simulink model "OcularMotorLabModel_2024_01_02_M21b"  (R2021b)
settings: Solver=FixedStepAuto  StartTime=tStart  StopTime=tFinal  FixedStep=0.001  RelTol=1e-3
undefined symbols (not defined in the file or in its folder): Asp, Asp1, Asp2, e0sp, gaussian, Gpc, GPos, Gsl, HeadToEye, IPD, psi, Psp1, RotFbk, SacThDeg, SatSp, sigbuilder_block, SomFbk, T1, T2, Tccanal, Tcn, Tcr, Tcsp, TCvs, tdm, tdsp1, tdsp2, tdsp3, tdv, Tsl, Tz, w
libraries: matrix_library x16, vrlib x9, simulink_extras x8, simulink x1
(part 2 of 2)

== system OcularMotorLabModel_2024_01_02_M21b/Right eye plant ==
  In1 : Inport
  Demux : Demux  Outputs=3
  Mux : Mux  Inputs=3
  Plant1 : TransferFcn  Numerator=[Tz 1]  Denominator=[T1*T2 (T1+T2) 1]
  Plant2 : TransferFcn  Numerator=[w^2]  Denominator=[1 + 2*psi*w w^2]
  Plant3 : TransferFcn  Numerator=[Tz 1]  Denominator=[T1*T2 (T1+T2) 1]
  Plant4 : TransferFcn  Numerator=[w^2]  Denominator=[1 + 2*psi*w w^2]
  Plant5 : TransferFcn  Numerator=[Tz 1]  Denominator=[T1*T2 (T1+T2) 1]
  Plant6 : TransferFcn  Numerator=[w^2]  Denominator=[1 + 2*psi*w w^2]
  Saturation : Saturate  UpperLimit=50*pi/180  LowerLimit=-50*pi/180
  Eye position : Outport
  wires:
  In1/1 -> Demux/1
  Mux/1 -> Saturation/1  "Eye position"
  Plant4/1 -> Mux/1
  Plant2/1 -> Mux/2
  Plant6/1 -> Mux/3
  Demux/1 -> Plant3/1
  Demux/2 -> Plant1/1
  Demux/3 -> Plant5/1
  Saturation/1 -> Eye position/1
  Plant3/1 -> Plant4/1
  Plant1/1 -> Plant2/1
  Plant5/1 -> Plant6/1

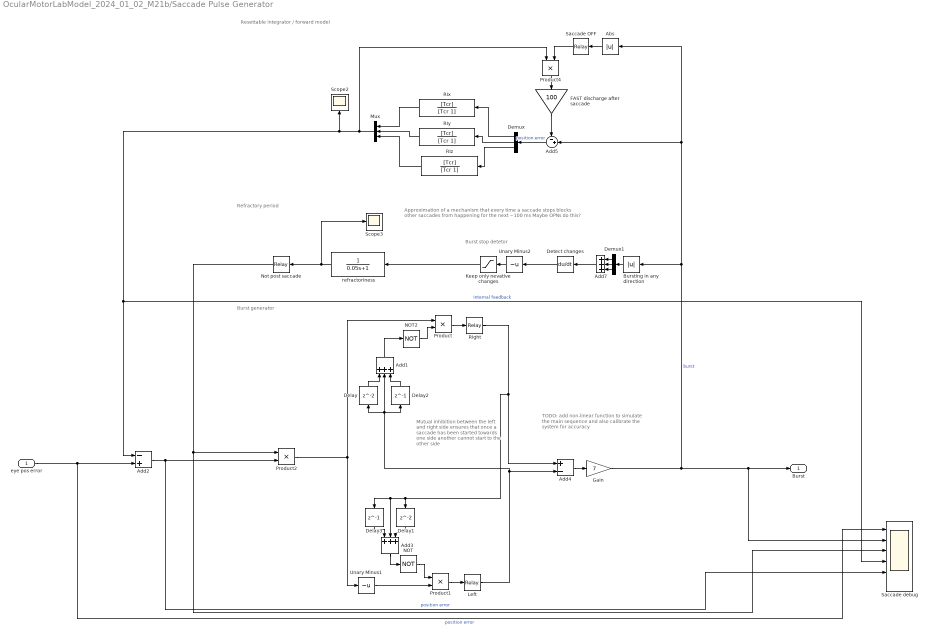
== system OcularMotorLabModel_2024_01_02_M21b/Saccade Pulse Generator ==
  note: Burst generator
  note: Resettable integrator / forward model
  note: Refractory period
  note: Burst stop detetor
  note: Mutual inhibition between the left and right side ensures that once a saccade has been started towards one side another cannot start to the other side
  note: TODO: add non-linear function to simulate the main sequence and also calibrate the system for accuracy
  note: Approximation of a mechanism that every time a saccade stops blocks other saccades from happening for the next ~100 ms
      | Maybe OPNs do this?
  eye pos error : Inport
  Abs : Abs
  Add1 : Sum  Inputs=+++
  Add2 : Sum  Inputs=-+
  Add3 : Sum  Inputs=+++
  Add4 : Sum  Inputs=+-
  Add5 : Sum  Inputs=-+|
  Add7 : Sum  Inputs=+++
  Bursting in any direction : Abs
  Delay : Delay  InitialCondition=0
  Delay1 : Delay  InitialCondition=0
  Delay2 : Delay  DelayLength=1  InitialCondition=0
  Delay3 : Delay  DelayLength=1  InitialCondition=0
  Demux : Demux  Outputs=3
  Demux1 : Demux  Outputs=3
  Detect changes : Derivative
  FAST discharge after saccade : Gain  Gain=100
  Gain : Gain  Gain=7
  Keep only nevative changes : Saturate  UpperLimit=50000000  LowerLimit=0
  Left : Relay  OnSwitchValue=SacThDeg/180*pi  OffSwitchValue=0
  Mux : Mux  Inputs=3
  NOT : Logic  Operator=NOT  IconShape=distinctive  AllPortsSameDT=off  OutDataTypeStr=boolean
  NOT2 : Logic  Operator=NOT  IconShape=distinctive  AllPortsSameDT=off  OutDataTypeStr=boolean
  Not post saccade : Relay  OnSwitchValue=1  OffSwitchValue=1  OnOutputValue=0  OffOutputValue=1
  Product{,1..2,4} (4 alike) : Product
  RIx : TransferFcn  Numerator=[Tcr]  Denominator=[Tcr 1]
  RIy : TransferFcn  Numerator=[Tcr]  Denominator=[Tcr 1]
  RIz : TransferFcn  Numerator=[Tcr]  Denominator=[Tcr 1]
  Right : Relay  OnSwitchValue=SacThDeg/180*pi  OffSwitchValue=0
  Saccade OFF : Relay  OnOutputValue=0  OffOutputValue=1
  Saccade debug : Scope  NumInputPorts=6
  Scope2 : Scope
  Scope3 : Scope
  Unary Minus1 : UnaryMinus
  Unary Minus2 : UnaryMinus
  refractoriness : TransferFcn  Numerator=1  Denominator=[0.05 1]
  Burst : Outport  VectorParamsAs1DForOutWhenUnconnected=off
  wires:
  eye pos error/1 -> Saccade debug/1, Add2/2  "position error"
  Add2/1 -> Saccade debug/5, Product2/2  "position error"
  Add7/1 -> Detect changes/1
  Detect changes/1 -> Unary Minus2/1
  Demux1/1 -> Add7/1
  Demux1/3 -> Add7/3
  Unary Minus2/1 -> Keep only nevative changes/1
  Demux1/2 -> Add7/2
  Bursting in any direction/1 -> Demux1/1
  refractoriness/1 -> Not post saccade/1, Scope3/1
  Keep only nevative changes/1 -> refractoriness/1
  Abs/1 -> Saccade OFF/1
  Product4/1 -> FAST discharge after saccade/1
  Mux/1 -> Saccade debug/4, Add2/1, Scope2/1, Product4/1  "Internal feedback"
  FAST discharge after saccade/1 -> Add5/1
  Saccade OFF/1 -> Product4/2
  Not post saccade/1 -> Saccade debug/3, Product2/1
  Add3/1 -> NOT/1
  Delay/1 -> Add1/1
  Delay2/1 -> Add1/3
  Unary Minus1/1 -> Product1/2
  Add4/1 -> Gain/1
  Product2/1 -> Product/1, Unary Minus1/1
  Add1/1 -> NOT2/1
  Product1/1 -> Left/1
  Product/1 -> Right/1
  NOT2/1 -> Product/2
  Delay1/1 -> Add3/3
  NOT/1 -> Product1/1
  Left/1 -> Add4/2, Delay2/1, Add1/2, Delay/1
  Gain/1 -> Saccade debug/2, Burst/1, Abs/1, Add5/2, Bursting in any direction/1  "burst"
  Delay3/1 -> Add3/1
  Right/1 -> Delay3/1, Add3/2, Delay1/1, Add4/1
  Demux/1 -> RIx/1
  RIy/1 -> Mux/2
  RIx/1 -> Mux/1
  Demux/3 -> RIz/1
  Demux/2 -> RIy/1
  RIz/1 -> Mux/3
  Add5/1 -> Demux/1  "position error"

== system OcularMotorLabModel_2024_01_02_M21b/Saccade velocity corollary ==
  note: Gaze holding integrator
  note: It's important for this internal model to not have a leaky integrator. Otherwise a positive feedback loop is created with retinal motion that it is not discounted but amplified post saccades.
      |
      | Haven't fully grasped it and there are still questions about the plant and the slide. But for now this seems to work ok.
  Burst : Inport
  Corollary debug : Scope  NumInputPorts=6
  Demux2 : Demux  Outputs=3
  Direct : Gain  Gain=Gpc
  Eye plant : Subsystem
  Integrator : Integrator
  "MN " : Sum  Inputs=+++  InputSameDT=on  SaturateOnIntegerOverflow=on  OutDataTypeStr=Inherit: Same as first input
  Mux2 : Mux  Inputs=3
  Pos2Vel1 : Derivative
  Position bias6 : TransferFcn  Numerator=[Gsl]  Denominator=[Tsl 1]
  Position bias7 : TransferFcn  Numerator=[Gsl]  Denominator=[Tsl 1]
  Position bias8 : TransferFcn  Numerator=[Gsl]  Denominator=[Tsl 1]
  Transport Delay : TransportDelay  DelayTime=tdv+tdm
  Out1 : Outport
  wires:
  Burst/1 -> Integrator/1, Direct/1, Demux2/1, Corollary debug/1  "Corollary input"
  Eye plant/1(Eye position) -> Pos2Vel1/1, Corollary debug/3  "Corollary eye position"
  "MN "/1 -> Eye plant/1(In1), Corollary debug/4  "Corollary integrator"
  Transport Delay/1 -> Out1/1
  Pos2Vel1/1 -> Corollary debug/2, Transport Delay/1  "Corollary eye velocity"
  Mux2/1 -> "MN "/3
  Integrator/1 -> "MN "/1
  Demux2/2 -> Position bias7/1
  Position bias8/1 -> Mux2/3
  Demux2/3 -> Position bias8/1
  Position bias6/1 -> Mux2/1
  Demux2/1 -> Position bias6/1
  Position bias7/1 -> Mux2/2
  Direct/1 -> "MN "/2

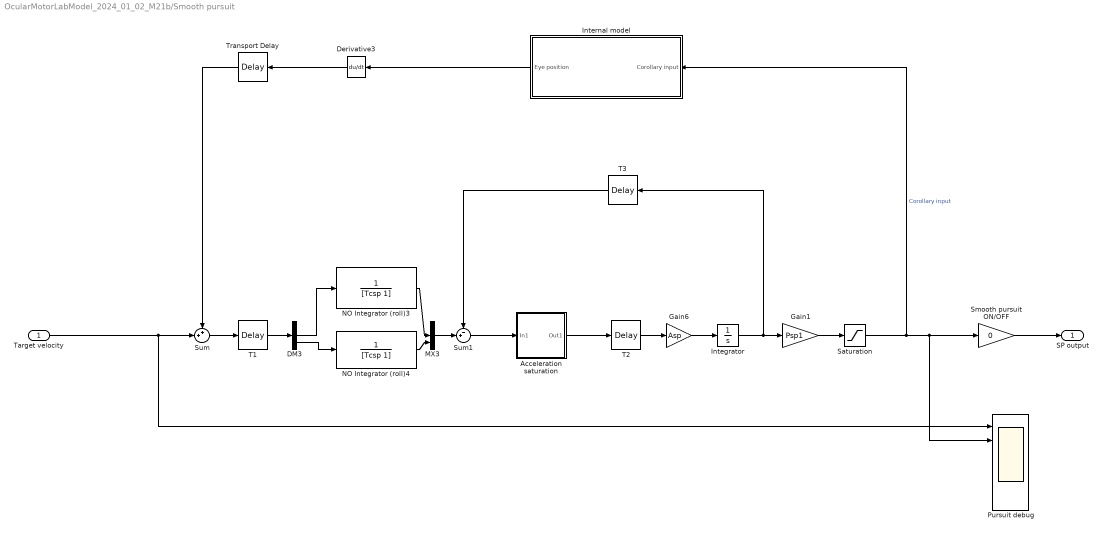
== system OcularMotorLabModel_2024_01_02_M21b/Smooth pursuit ==
  Target velocity : Inport
  Acceleration saturation : Subsystem
  DM3 : Demux  Outputs=3
  Derivative3 : Derivative
  Gain1 : Gain  Gain=Psp1
  Gain6 : Gain  Gain=Asp
  Integrator : Integrator
  Internal model : Subsystem
  MX3 : Mux  Inputs=3
  NO Integrator (roll)3 : TransferFcn  Denominator=[Tcsp 1]
  NO Integrator (roll)4 : TransferFcn  Denominator=[Tcsp 1]
  Pursuit debug : Scope  NumInputPorts=6
  Saturation : Saturate  UpperLimit=deg2rad(SatSp)  LowerLimit=-deg2rad(SatSp)
  Smooth pursuit ON/OFF : Gain  Gain=0
  Sum : Sum  Inputs=++|
  Sum1 : Sum  Inputs=-+|
  T1 : TransportDelay  DelayTime=tdsp1
  T2 : TransportDelay  DelayTime=tdsp2
  T3 : TransportDelay  DelayTime=tdsp3
  Transport Delay : TransportDelay  DelayTime=tdv+tdm
  SP output : Outport
  wires:
  Target velocity/1 -> Pursuit debug/1, Sum/2
  Sum/1 -> T1/1
  Transport Delay/1 -> Sum/1
  MX3/1 -> Sum1/2
  DM3/2 -> NO Integrator (roll)3/1
  NO Integrator (roll)3/1 -> MX3/2
  DM3/3 -> NO Integrator (roll)4/1
  NO Integrator (roll)4/1 -> MX3/3
  T1/1 -> DM3/1
  Gain6/1 -> Integrator/1
  Integrator/1 -> T3/1, Gain1/1
  T2/1 -> Gain6/1
  T3/1 -> Sum1/1
  Gain1/1 -> Saturation/1
  Smooth pursuit ON/OFF/1 -> SP output/1
  Saturation/1 -> Internal model/1(Corollary input), Pursuit debug/2, Smooth pursuit ON/OFF/1  "Corollary input"
  Derivative3/1 -> Transport Delay/1
  Internal model/1(Eye position) -> Derivative3/1
  Sum1/1 -> Acceleration saturation/1(In1)
  Acceleration saturation/1(Out1) -> T2/1

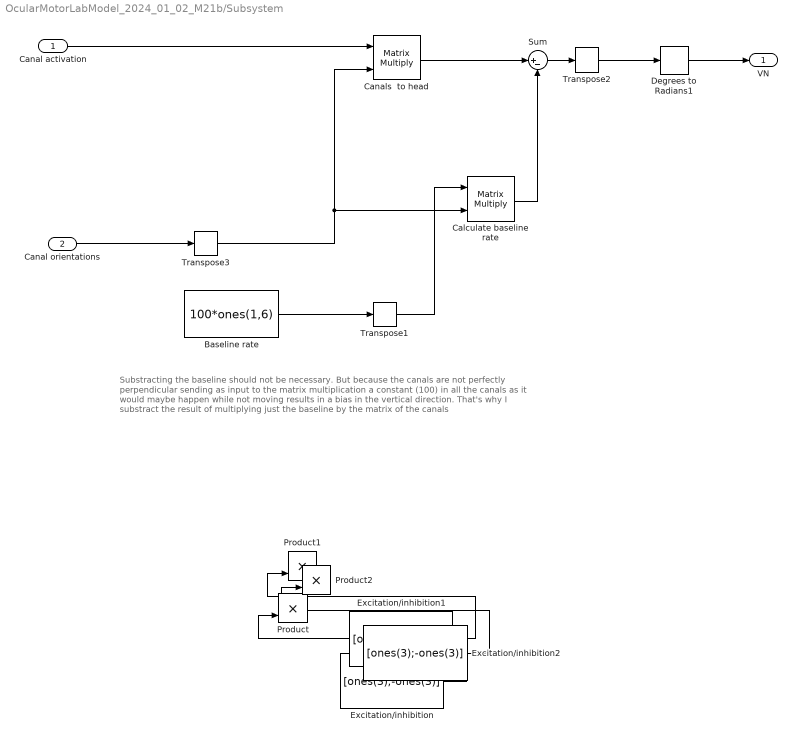
== system OcularMotorLabModel_2024_01_02_M21b/Subsystem ==
  note: Substracting the baseline should not be necessary. But because the canals are not perfectly perpendicular sending as input to the matrix multiplication a constant (100) in all the canals as it would maybe happen while not moving results in a bias in the vertical direction. That's why I substract the result of multiplying just the baseline by the matrix of the canals
  Canal activation : Inport
  Canal orientations : Inport  Port=2
  Baseline rate : Constant  Value=100*ones(1,6)
  Calculate baseline rate : Product  Multiplication=Matrix(*)
  Canals  to head : Product  Multiplication=Matrix(*)
  Degrees to Radians1 : simulink_extras/Transformations/Degrees to Radians
  Excitation/inhibition : Constant  Value=[ones(3);-ones(3)]  VectorParams1D=off
  Excitation/inhibition1 : Constant  Value=[ones(3);-ones(3)]  VectorParams1D=off
  Excitation/inhibition2 : Constant  Value=[ones(3);-ones(3)]  VectorParams1D=off
  Product : Product
  Product1 : Product
  Product2 : Product
  Sum : Sum  Inputs=|+-
  Transpose1 : matrix_library/Transpose
  Transpose2 : matrix_library/Transpose
  Transpose3 : matrix_library/Transpose
  VN : Outport
  wires:
  Sum/1 -> Transpose2/1
  Transpose2/1 -> Degrees to Radians1/1
  Transpose3/1 -> Calculate baseline rate/2, Canals  to head/2
  Excitation/inhibition/1 -> Product/2
  Excitation/inhibition1/1 -> Product1/2
  Excitation/inhibition2/1 -> Product2/2
  Canal orientations/1 -> Transpose3/1
  Canal activation/1 -> Canals  to head/1
  Baseline rate/1 -> Transpose1/1
  Calculate baseline rate/1 -> Sum/2
  Canals  to head/1 -> Sum/1
  Transpose1/1 -> Calculate baseline rate/1
  Degrees to Radians1/1 -> VN/1

== system OcularMotorLabModel_2024_01_02_M21b/Target position ==
  Bus Creator : BusCreator  Tag=Bus Creator  Inputs=3
  FromWs : FromWorkspace  Tag=STV FromWs  VariableName=tuvar
      SigBuilderData=|
      | common.afterFinalStr = 'Extrapolate'
      | common.sampleTime = 0
      | dataSet(1).timeRange = [0 88]
      | dataSet(1).name = 'Fixed streight ahead'
      | dataSet(2).timeRange = [0 88]
      | dataSet(2).name = 'Saccade Left and back'
      | dataSet(3).timeRange = [0 88]
      | dataSet(3).name = 'Saccade Right and back small'
      | dataSet(4).timeRange = [0 88]
      | dataSet(4).name = 'Saccade Up down and back'
      | dataSet(5).timeRange = [0 88]
      | dataSet(5).name = 'Horizontal smooth pursuit'
      | dataSet(6).timeRange = [0 88]
      | dataSet(6).name = 'Vergence'
      | dataSet(7).timeRange = [0 88]
      | dataSet(7).name = 'Saccade Oblique'
      | sbobj.Groups(1).Name = 'Fixed streight ahead'
      | sbobj.Groups(1).Signals(1).Name = 'tX (m - postiive forward)'
      | sbobj.Groups(1).Signals(1).XData = [0 88]
      | sbobj.Groups(1).Signals(1).YData = [1 1]
      | sbobj.Groups(1).Signals(2).Name = 'tY (m - postive to left)'
      | sbobj.Groups(1).Signals(2).XData = [0 5 35 88]
      | sbobj.Groups(1).Signals(2).YData = [0 0 0 0]
      | sbobj.Groups(1).Signals(3).Name = 'tZ (m - positive up)'
      | sbobj.Groups(1).Signals(3).XData = [0 88]
      | sbobj.Groups(1).Signals(3).YData = [0 0]
      | sbobj.Groups(1).TimeRange = [0 88]
      | sbobj.Groups(2).Name = 'Saccade Left and back'
      | sbobj.Groups(2).Signals(1).Name = 'tX (m - postiive forward)'
      | sbobj.Groups(2).Signals(1).XData = [0 88]
      | sbobj.Groups(2).Signals(1).YData = [1 1]
      | sbobj.Groups(2).Signals(2).Name = 'tY (m - postive to left)'
      | sbobj.Groups(2).Signals(2).XData = [0 5 5 25.1 25.1 88]
      | sbobj.Groups(2).Signals(2).YData = [0 0 0.5 0.5 0 0]
      | sbobj.Groups(2).Signals(3).Name = 'tZ (m - positive up)'
      | sbobj.Groups(2).Signals(3).XData = [0 88]
      | sbobj.Groups(2).Signals(3).YData = [0 0]
      | sbobj.Groups(2).TimeRange = [0 88]
      | sbobj.Groups(3).Name = 'Saccade Right and back small'
      | sbobj.Groups(3).Signals(1).Name = 'tX (m - postiive forward)'
      | sbobj.Groups(3).Signals(1).XData = [0 88]
      | sbobj.Groups(3).Signals(1).YData = [1 1]
      | sbobj.Groups(3).Signals(2).Name = 'tY (m - postive to left)'
      | sbobj.Groups(3).Signals(2).XData = [0 5 5 35 35 88]
      | sbobj.Groups(3).Signals(2).YData = [0 0 0.02 0.02 0 0]
      | sbobj.Groups(3).Signals(3).Name = 'tZ (m - positive up)'
      | sbobj.Groups(3).Signals(3).XData = [0 88]
      | sbobj.Groups(3).Signals(3).YData = [0 0]
      | sbobj.Groups(3).TimeRange = [0 88]
      | sbobj.Groups(4).Name = 'Saccade Up down and back'
      | sbobj.Groups(4).Signals(1).Name = 'tX (m - postiive forward)'
      | sbobj.Groups(4).Signals(1).XData = [0 88]
      | sbobj.Groups(4).Signals(1).YData = [1 1]
      | sbobj.Groups(4).Signals(2).Name = 'tY (m - postive to left)'
      | sbobj.Groups(4).Signals(2).XData = [0 5 35 88]
      | sbobj.Groups(4).Signals(2).YData = [0 0 0 0]
      | sbobj.Groups(4).Signals(3).Name = 'tZ (m - positive up)'
      | sbobj.Groups(4).Signals(3).XData = [0 10 10 13.1 13.1 88]
      | sbobj.Groups(4).Signals(3).YData = [0 0 0.5 0.5 0 0]
      | sbobj.Groups(4).TimeRange = [0 88]
      | sbobj.Groups(5).Name = 'Horizontal smooth pursuit'
      | sbobj.Groups(5).Signals(1).Name = 'tX (m - postiive forward)'
      | sbobj.Groups(5).Signals(1).XData = [0 88]
      | sbobj.Groups(5).Signals(1).YData = [1 1]
      | sbobj.Groups(5).Signals(2).Name = 'tY (m - postive to left)'
      | sbobj.Groups(5).Signals(2).XData = [0 10 20 20 88]
      | sbobj.Groups(5).Signals(2).YData = [0 0 0.5 0 0]
      | sbobj.Groups(5).Signals(3).Name = 'tZ (m - positive up)'
      | sbobj.Groups(5).Signals(3).XData = [0 10 20 88]
      | sbobj.Groups(5).Signals(3).YData = [0 0 0 0]
      | sbobj.Groups(5).TimeRange = [0 88]
      | sbobj.Groups(6).Name = 'Vergence'
      | sbobj.Groups(6).Signals(1).Name = 'tX (m - postiive forward)'
      | sbobj.Groups(6).Signals(1).XData = [0 10 10 20 20 30 30 40 40 50 50 60 60 70 70 80 80 88]
      | sbobj.Groups(6).Signals(1).YData = [1.25 1.25 0.25 0.25 1.25 1.25 0.25 0.25 1.25 1.25 0.25 0.25 1.25 1.25 0.25 0.25 1.25 1.25]
      | sbobj.Groups(6).Signals(2).Name = 'tY (m - postive to left)'
      | sbobj.Groups(6).Signals(2).XData = [0 5 25.1 88]
      | sbobj.Groups(6).Signals(2).YData = [0 0 0 0]
      | sbobj.Groups(6).Signals(3).Name = 'tZ (m - positive up)'
      | sbobj.Groups(6).Signals(3).XData = [0 88]
      | sbobj.Groups(6).Signals(3).YData = [0 0]
      | sbobj.Groups(6).TimeRange = [0 88]
      | sbobj.Groups(7).Name = 'Saccade Oblique'
      | sbobj.Groups(7).Signals(1).Name = 'tX (m - postiive forward)'
      | sbobj.Groups(7).Signals(1).XData = [0 88]
      | sbobj.Groups(7).Signals(1).YData = [1 1]
      | sbobj.Groups(7).Signals(2).Name = 'tY (m - postive to left)'
      | sbobj.Groups(7).Signals(2).XData = [0 10 10 20 20 88]
      | sbobj.Groups(7).Signals(2).YData = [0 0 0.5 0.5 0 0]
      | sbobj.Groups(7).Signals(3).Name = 'tZ (m - positive up)'
      | sbobj.Groups(7).Signals(3).XData = [0 10 10 20 20 88]
      | sbobj.Groups(7).Signals(3).YData = [0 0 0.5 0.5 0 0]
      | sbobj.Groups(7).TimeRange = [0 88]
  Subsystem : Subsystem
  Bus : Outport
  wires:
  FromWs/1 -> Subsystem/1(In1)
  Subsystem/1(tX (m - postiive forward)) -> Bus Creator/1  "tX (m - postiive forward)"
  Subsystem/2(tY (m - postive to left)) -> Bus Creator/2  "tY (m - postive to left)"
  Subsystem/3(tZ (m - positive up)) -> Bus Creator/3  "tZ (m - positive up)"
  Bus Creator/1 -> Bus/1

== system OcularMotorLabModel_2024_01_02_M21b/Velocity storage ==
  In1 : Inport
  DM : Demux  Outputs=3
  IA Integrator (pitch) : TransferFcn  Numerator=1  Denominator=[TCvs 1]
  MX : Mux  Inputs=3
  NO Integrator (roll) : TransferFcn  Numerator=1  Denominator=[TCvs 1]
  RC Integrator (yaw) : TransferFcn  Numerator=1  Denominator=[TCvs 1]
  Out1 : Outport
  wires:
  MX/1 -> Out1/1
  DM/3 -> RC Integrator (yaw)/1
  RC Integrator (yaw)/1 -> MX/3
  IA Integrator (pitch)/1 -> MX/2
  NO Integrator (roll)/1 -> MX/1
  DM/1 -> NO Integrator (roll)/1
  In1/1 -> DM/1
  DM/2 -> IA Integrator (pitch)/1

== system OcularMotorLabModel_2024_01_02_M21b/Vergence ==
  Target distance estimate (Diopters) : Inport
  Vergence error : Inport  Port=2
  Transfer Fcn : TransferFcn  Denominator=[0.1 1]
  Vergence on/off : Gain
  Vergence : Outport
  Accomodation : Outport  Port=2
  wires:
  Vergence on/off/1 -> Vergence/1
  Vergence error/1 -> Transfer Fcn/1
  Target distance estimate (Diopters)/1 -> ?
  Transfer Fcn/1 -> Vergence on/off/1

== system OcularMotorLabModel_2024_01_02_M21b/Vergence (distance) corollary ==
  Motor output : Inport
  Asin5 : Trigonometry  Operator=tan
  Corollary debug : Scope  NumInputPorts=6
  Divide3 : Product  Inputs=*/
  Eye plant : Subsystem
  IPD : Constant  Value=IPD/2
  Diopters : Outport
  wires:
  Motor output/1 -> Corollary debug/1, Eye plant/1(Motor output)  "Corollary input"
  Eye plant/1(Eye position) -> Corollary debug/2, Asin5/1  "Corollary eye position"
  Divide3/1 -> Diopters/1, Corollary debug/3
  IPD/1 -> Divide3/2
  Asin5/1 -> Divide3/1

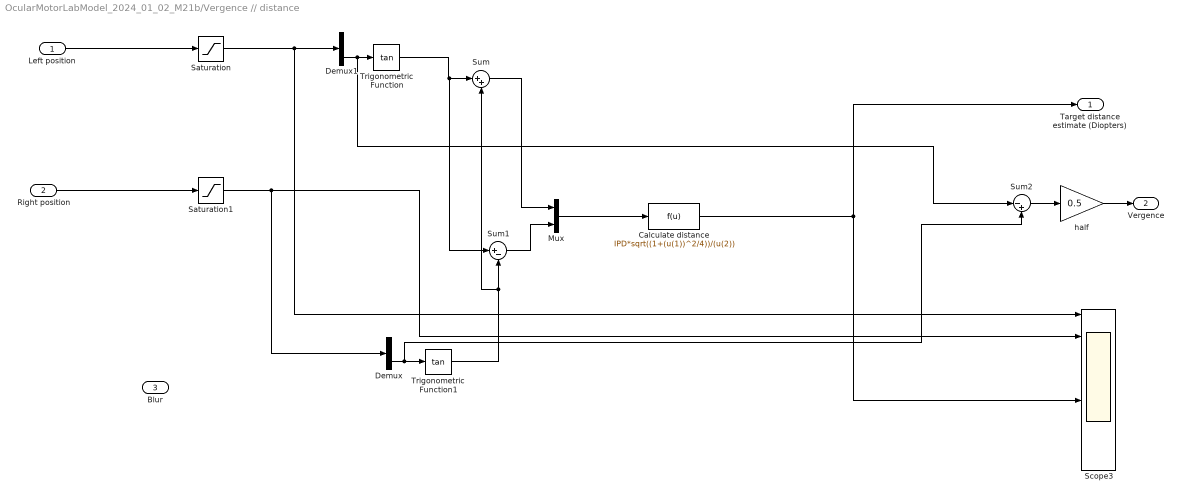
== system OcularMotorLabModel_2024_01_02_M21b/Vergence // distance ==
  Left position : Inport
  Right position : Inport  Port=2
  Blur : Inport  Port=3
  Calculate distance : Fcn  Expr=IPD*sqrt((1+(u(1))^2/4))/(u(2))
  Demux : Demux  Outputs=3
  Demux1 : Demux  Outputs=3
  Mux : Mux  Inputs=2
  Saturation : Saturate  UpperLimit=50*pi/180  LowerLimit=-50*pi/180
  Saturation1 : Saturate  UpperLimit=50*pi/180  LowerLimit=-50*pi/180
  Scope3 : Scope  NumInputPorts=8
  Sum : Sum  Inputs=|++
  Sum1 : Sum  Inputs=|+-
  Sum2 : Sum  Inputs=|-+
  Trigonometric Function : Trigonometry  Operator=tan
  Trigonometric Function1 : Trigonometry  Operator=tan
  half : Gain  Gain=0.5
  Target distance estimate (Diopters) : Outport
  Vergence : Outport  Port=2
  wires:
  Left position/1 -> Saturation/1
  Right position/1 -> Saturation1/1
  Mux/1 -> Calculate distance/1
  Demux1/3 -> Sum2/1, Trigonometric Function/1
  Demux/3 -> Sum2/2, Trigonometric Function1/1
  Calculate distance/1 -> Scope3/5, Target distance estimate (Diopters)/1
  Trigonometric Function/1 -> Sum1/1, Sum/1
  Trigonometric Function1/1 -> Sum/2, Sum1/2
  Sum/1 -> Mux/1
  Sum1/1 -> Mux/2
  Sum2/1 -> half/1
  Saturation/1 -> Scope3/1, Demux1/1
  Saturation1/1 -> Scope3/2, Demux/1
  half/1 -> Vergence/1

== system OcularMotorLabModel_2024_01_02_M21b/Version ==
  Left : Inport
  Right : Inport  Port=2
  Gain : Gain  Gain=1/2
  Saccade debug : Scope  NumInputPorts=6
  Sum : Sum  Inputs=+|+
  Out1 : Outport
  wires:
  Gain/1 -> Saccade debug/3, Out1/1
  Sum/1 -> Gain/1
  Left/1 -> Saccade debug/1, Sum/1
  Right/1 -> Saccade debug/2, Sum/2

== system OcularMotorLabModel_2024_01_02_M21b/Version Position corollary ==
  Motor output : Inport
  Asin1 : Trigonometry
  Asin2 : Trigonometry  Operator=cos
  Asin3 : Trigonometry  Operator=cos
  Asin4 : Trigonometry
  Corollary debug : Scope  NumInputPorts=6
  Demux3 : Demux  Outputs=3
  Divide1 : Product  Inputs=**
  Divide2 : Product  Inputs=**
  Eye plant : Subsystem
  Mux3 : Mux  Inputs=3
  Out1 : Outport
  wires:
  Eye plant/1(Eye position) -> Demux3/1, Corollary debug/3  "Corollary eye position"
  Divide1/1 -> Mux3/1
  Asin1/1 -> Mux3/3
  Demux3/2 -> Asin3/1, Asin1/1
  Divide2/1 -> Mux3/2
  Asin3/1 -> Divide2/2, Divide1/2
  Asin2/1 -> Divide1/1
  Asin4/1 -> Divide2/1
  Demux3/3 -> Asin2/1, Asin4/1
  Mux3/1 -> Corollary debug/5, Out1/1  "Step"
  Motor output/1 -> Eye plant/1(Motor output)  "Corollary input"

== system OcularMotorLabModel_2024_01_02_M21b/Visual World Extrinsic Orientation ==
  Bus Creator : BusCreator  Tag=Bus Creator  Inputs=3
  FromWs : FromWorkspace  Tag=STV FromWs  VariableName=tuvar
      SigBuilderData=|
      | common.afterFinalStr = 'Extrapolate'
      | common.sampleTime = 0
      | dataSet(1).timeRange = [0 60]
      | dataSet(1).name = 'Zeros'
      | dataSet(2).timeRange = [0 60]
      | dataSet(2).name = 'Roll 0.2 Hz'
      | dataSet(3).timeRange = [0 60]
      | dataSet(3).name = 'Roll 0.1 Hz'
      | dataSet(4).timeRange = [0 60]
      | dataSet(4).name = 'Roll 0.05 Hz'
      | dataSet(5).timeRange = [0 60]
      | dataSet(5).name = 'Roll 0.2 Hz IA'
      | dataSet(6).timeRange = [0 60]
      | dataSet(6).name = 'Roll 0.1 Hz IA'
      | dataSet(7).timeRange = [0 60]
      | dataSet(7).name = 'Roll 0.05 Hz IA'
      | dataSet(8).timeRange = [0 60]
      | dataSet(8).name = 'Roll 0.2 Hz RC'
      | dataSet(9).timeRange = [0 60]
      | dataSet(9).name = 'Roll 0.1 Hz RC'
      | dataSet(10).timeRange = [0 60]
      | dataSet(10).name = 'Roll 0.05 Hz RC'
      | dataSet(11).timeRange = [0 60]
      | dataSet(11).name = 'SimpleSims'
      | sbobj.Groups(1).Name = 'Zeros'
      | sbobj.Groups(1).Signals(1).Name = 'N-O (roll)'
      | sbobj.Groups(1).Signals(1).XData = [0 60]
      | sbobj.Groups(1).Signals(1).YData = [0 0]
      | sbobj.Groups(1).Signals(2).Name = 'I-A (pitch)'
      | sbobj.Groups(1).Signals(2).XData = [0 60]
      | sbobj.Groups(1).Signals(2).YData = [0 0]
      | sbobj.Groups(1).Signals(3).Name = 'R-C (yaw)'
      | sbobj.Groups(1).Signals(3).XData = [0 60]
      | sbobj.Groups(1).Signals(3).YData = [0 0]
      | sbobj.Groups(1).TimeRange = [0 60]
      | sbobj.Groups(2).Name = 'Roll 0.2 Hz'
      | sbobj.Groups(2).Signals(1).Name = 'N-O (roll)'
      | sbobj.Groups(2).Signals(1).XData = [0 0.00500500500501 0.01001001001 0.015015015015 0.02002002002 0.025025025025 0.03003003003 0.035035035035 0.04004004004 0.045045045045 0.0500500500501 0.0550550550551 ... (11989 elements, 1x11989)]
      | sbobj.Groups(2).Signals(1).YData = [0 0.125788666321 0.251572356775 0.377346095689 0.503104907788 0.628843818382 0.754557853574 0.880242040448 1.00589140727 1.13150098368 1.25706580089 1.3825808919 ... (11989 elements, 1x11989)]
      | sbobj.Groups(2).Signals(2).Name = 'I-A (pitch)'
      | sbobj.Groups(2).Signals(2).XData = [0 60]
      | sbobj.Groups(2).Signals(2).YData = [0 0]
      | sbobj.Groups(2).Signals(3).Name = 'R-C (yaw)'
      | sbobj.Groups(2).Signals(3).XData = [0 60]
      | sbobj.Groups(2).Signals(3).YData = [0 0]
      | sbobj.Groups(2).TimeRange = [0 60]
      | sbobj.Groups(3).Name = 'Roll 0.1 Hz'
      | sbobj.Groups(3).Signals(1).Name = 'N-O (roll)'
      | sbobj.Groups(3).Signals(1).XData = [0 0.01001001001 0.02002002002 0.03003003003 0.04004004004 0.0500500500501 0.0600600600601 0.0700700700701 0.0800800800801 0.0900900900901 0.1001001001 0.11011011011 ... (5995 elements, 1x5995)]
      | sbobj.Groups(3).Signals(1).YData = [0 0.125788666321 0.251572356775 0.377346095689 0.503104907788 0.628843818382 0.754557853574 0.880242040448 1.00589140727 1.13150098368 1.25706580089 1.3825808919 ... (5995 elements, 1x5995)]
      | sbobj.Groups(3).Signals(2).Name = 'I-A (pitch)'
      | sbobj.Groups(3).Signals(2).XData = [0 60]
      | sbobj.Groups(3).Signals(2).YData = [0 0]
      | sbobj.Groups(3).Signals(3).Name = 'R-C (yaw)'
      | sbobj.Groups(3).Signals(3).XData = [0 60]
      | sbobj.Groups(3).Signals(3).YData = [0 0]
      | sbobj.Groups(3).TimeRange = [0 60]
      | sbobj.Groups(4).Name = 'Roll 0.05 Hz'
      | sbobj.Groups(4).Signals(1).Name = 'N-O (roll)'
      | sbobj.Groups(4).Signals(1).XData = [0 0.02002002002 0.04004004004 0.0600600600601 0.0800800800801 0.1001001001 0.12012012012 0.14014014014 0.16016016016 0.18018018018 0.2002002002 0.22022022022 ... (2998 elements, 1x2998)]
      | sbobj.Groups(4).Signals(1).YData = [0 0.125788666321 0.251572356775 0.377346095689 0.503104907788 0.628843818382 0.754557853574 0.880242040448 1.00589140727 1.13150098368 1.25706580089 1.3825808919 ... (2998 elements, 1x2998)]
      | sbobj.Groups(4).Signals(2).Name = 'I-A (pitch)'
      | sbobj.Groups(4).Signals(2).XData = [0 60]
      | sbobj.Groups(4).Signals(2).YData = [0 0]
      | sbobj.Groups(4).Signals(3).Name = 'R-C (yaw)'
      | sbobj.Groups(4).Signals(3).XData = [0 60]
      | sbobj.Groups(4).Signals(3).YData = [0 0]
      | sbobj.Groups(4).TimeRange = [0 60]
      | sbobj.Groups(5).Name = 'Roll 0.2 Hz IA'
      | sbobj.Groups(5).Signals(1).Name = 'N-O (roll)'
      | sbobj.Groups(5).Signals(1).XData = [0 60]
      | sbobj.Groups(5).Signals(1).YData = [0 0]
      | sbobj.Groups(5).Signals(2).Name = 'I-A (pitch)'
      | sbobj.Groups(5).Signals(2).XData = [0 0.00500500500501 0.01001001001 0.015015015015 0.02002002002 0.025025025025 0.03003003003 0.035035035035 0.04004004004 0.045045045045 0.0500500500501 0.0550550550551 ... (11989 elements, 1x11989)]
      | sbobj.Groups(5).Signals(2).YData = [0 0.125788666321 0.251572356775 0.377346095689 0.503104907788 0.628843818382 0.754557853574 0.880242040448 1.00589140727 1.13150098368 1.25706580089 1.3825808919 ... (11989 elements, 1x11989)]
      | sbobj.Groups(5).Signals(3).Name = 'R-C (yaw)'
      | sbobj.Groups(5).Signals(3).XData = [0 60]
      | sbobj.Groups(5).Signals(3).YData = [0 0]
      | sbobj.Groups(5).TimeRange = [0 60]
      | sbobj.Groups(6).Name = 'Roll 0.1 Hz IA'
      | sbobj.Groups(6).Signals(1).Name = 'N-O (roll)'
      | sbobj.Groups(6).Signals(1).XData = [0 60]
      | sbobj.Groups(6).Signals(1).YData = [0 0]
      | sbobj.Groups(6).Signals(2).Name = 'I-A (pitch)'
      | sbobj.Groups(6).Signals(2).XData = [0 0.01001001001 0.02002002002 0.03003003003 0.04004004004 0.0500500500501 0.0600600600601 0.0700700700701 0.0800800800801 0.0900900900901 0.1001001001 0.11011011011 ... (5995 elements, 1x5995)]
      | sbobj.Groups(6).Signals(2).YData = [0 0.125788666321 0.251572356775 0.377346095689 0.503104907788 0.628843818382 0.754557853574 0.880242040448 1.00589140727 1.13150098368 1.25706580089 1.3825808919 ... (5995 elements, 1x5995)]
      | sbobj.Groups(6).Signals(3).Name = 'R-C (yaw)'
      | sbobj.Groups(6).Signals(3).XData = [0 60]
      | sbobj.Groups(6).Signals(3).YData = [0 0]
      | sbobj.Groups(6).TimeRange = [0 60]
      | sbobj.Groups(7).Name = 'Roll 0.05 Hz IA'
      | sbobj.Groups(7).Signals(1).Name = 'N-O (roll)'
      | sbobj.Groups(7).Signals(1).XData = [0 60]
      | sbobj.Groups(7).Signals(1).YData = [0 0]
      | sbobj.Groups(7).Signals(2).Name = 'I-A (pitch)'
      | sbobj.Groups(7).Signals(2).XData = [0 0.02002002002 0.04004004004 0.0600600600601 0.0800800800801 0.1001001001 0.12012012012 0.14014014014 0.16016016016 0.18018018018 0.2002002002 0.22022022022 ... (2998 elements, 1x2998)]
      | sbobj.Groups(7).Signals(2).YData = [0 0.125788666321 0.251572356775 0.377346095689 0.503104907788 0.628843818382 0.754557853574 0.880242040448 1.00589140727 1.13150098368 1.25706580089 1.3825808919 ... (2998 elements, 1x2998)]
      | sbobj.Groups(7).Signals(3).Name = 'R-C (yaw)'
      | sbobj.Groups(7).Signals(3).XData = [0 60]
      | sbobj.Groups(7).Signals(3).YData = [0 0]
      | sbobj.Groups(7).TimeRange = [0 60]
      | sbobj.Groups(8).Name = 'Roll 0.2 Hz RC'
      | sbobj.Groups(8).Signals(1).Name = 'N-O (roll)'
      | sbobj.Groups(8).Signals(1).XData = [0 60]
      | sbobj.Groups(8).Signals(1).YData = [0 0]
      | sbobj.Groups(8).Signals(2).Name = 'I-A (pitch)'
      | sbobj.Groups(8).Signals(2).XData = [0 60]
      | sbobj.Groups(8).Signals(2).YData = [0 0]
      | sbobj.Groups(8).Signals(3).Name = 'R-C (yaw)'
      | sbobj.Groups(8).Signals(3).XData = [0 0.00500500500501 0.01001001001 0.015015015015 0.02002002002 0.025025025025 0.03003003003 0.035035035035 0.04004004004 0.045045045045 0.0500500500501 0.0550550550551 ... (11989 elements, 1x11989)]
      | sbobj.Groups(8).Signals(3).YData = [0 0.125788666321 0.251572356775 0.377346095689 0.503104907788 0.628843818382 0.754557853574 0.880242040448 1.00589140727 1.13150098368 1.25706580089 1.3825808919 ... (11989 elements, 1x11989)]
      | sbobj.Groups(8).TimeRange = [0 60]
      | sbobj.Groups(9).Name = 'Roll 0.1 Hz RC'
      | sbobj.Groups(9).Signals(1).Name = 'N-O (roll)'
      | sbobj.Groups(9).Signals(1).XData = [0 60]
      | sbobj.Groups(9).Signals(1).YData = [0 0]
      | sbobj.Groups(9).Signals(2).Name = 'I-A (pitch)'
      | sbobj.Groups(9).Signals(2).XData = [0 60]
      | sbobj.Groups(9).Signals(2).YData = [0 0]
      | sbobj.Groups(9).Signals(3).Name = 'R-C (yaw)'
      | sbobj.Groups(9).Signals(3).XData = [0 0.01001001001 0.02002002002 0.03003003003 0.04004004004 0.0500500500501 0.0600600600601 0.0700700700701 0.0800800800801 0.0900900900901 0.1001001001 0.11011011011 ... (5995 elements, 1x5995)]
      | sbobj.Groups(9).Signals(3).YData = [0 0.125788666321 0.251572356775 0.377346095689 0.503104907788 0.628843818382 0.754557853574 0.880242040448 1.00589140727 1.13150098368 1.25706580089 1.3825808919 ... (5995 elements, 1x5995)]
      | sbobj.Groups(9).TimeRange = [0 60]
      | sbobj.Groups(10).Name = 'Roll 0.05 Hz RC'
      | sbobj.Groups(10).Signals(1).Name = 'N-O (roll)'
      | sbobj.Groups(10).Signals(1).XData = [0 60]
      | sbobj.Groups(10).Signals(1).YData = [0 0]
      | sbobj.Groups(10).Signals(2).Name = 'I-A (pitch)'
      | sbobj.Groups(10).Signals(2).XData = [0 60]
      | sbobj.Groups(10).Signals(2).YData = [0 0]
      | sbobj.Groups(10).Signals(3).Name = 'R-C (yaw)'
      | sbobj.Groups(10).Signals(3).XData = [0 0.02002002002 0.04004004004 0.0600600600601 0.0800800800801 0.1001001001 0.12012012012 0.14014014014 0.16016016016 0.18018018018 0.2002002002 0.22022022022 ... (2998 elements, 1x2998)]
      | sbobj.Groups(10).Signals(3).YData = [0 0.125788666321 0.251572356775 0.377346095689 0.503104907788 0.628843818382 0.754557853574 0.880242040448 1.00589140727 1.13150098368 1.25706580089 1.3825808919 ... (2998 elements, 1x2998)]
      | sbobj.Groups(10).TimeRange = [0 60]
      | sbobj.Groups(11).Name = 'SimpleSims'
      | sbobj.Groups(11).Signals(1).Name = 'N-O (roll)'
      | sbobj.Groups(11).Signals(1).XData = [0 0.01 0.02 0.03 0.04 0.05 0.06 0.07 0.08 0.09 0.1 0.11 ... (6001 elements, 1x6001)]
      | sbobj.Groups(11).Signals(1).YData = [0 0.0628317497176 0.125662879311 0.188492768663 0.251320797667 0.314146346236 0.376968794308 0.43978752185 0.502601908867 0.565411335405 0.628215181563 0.691012827489 ... (6001 elements, 1x6001)]
      | sbobj.Groups(11).Signals(2).Name = 'I-A (pitch)'
      | sbobj.Groups(11).Signals(2).XData = [0 5 35 60]
      | sbobj.Groups(11).Signals(2).YData = [0 0 0 0]
      | sbobj.Groups(11).Signals(3).Name = 'R-C (yaw)'
      | sbobj.Groups(11).Signals(3).XData = [0 5 35 60]
      | sbobj.Groups(11).Signals(3).YData = [0 0 0 0]
      | sbobj.Groups(11).TimeRange = [0 60]
  Subsystem : Subsystem
  Bus : Outport
  wires:
  FromWs/1 -> Subsystem/1(In1)
  Subsystem/1(N-O (roll)) -> Bus Creator/1  "N-O (roll)"
  Subsystem/2(I-A (pitch)) -> Bus Creator/2  "I-A (pitch)"
  Subsystem/3(R-C (yaw)) -> Bus Creator/3  "R-C (yaw)"
  Bus Creator/1 -> Bus/1

== system OcularMotorLabModel_2024_01_02_M21b/Visual World Extrinsic velocity ==
  Bus Creator : BusCreator  Tag=Bus Creator  Inputs=3
  FromWs : FromWorkspace  Tag=STV FromWs  VariableName=tuvar
      SigBuilderData=|
      | common.afterFinalStr = 'Extrapolate'
      | common.sampleTime = 0
      | dataSet(1).timeRange = [0 60]
      | dataSet(1).name = 'Zeros'
      | dataSet(2).timeRange = [0 60]
      | dataSet(2).name = 'Roll 0.2 Hz'
      | dataSet(3).timeRange = [0 60]
      | dataSet(3).name = 'Roll 0.1 Hz'
      | dataSet(4).timeRange = [0 60]
      | dataSet(4).name = 'Roll 0.05 Hz'
      | dataSet(5).timeRange = [0 60]
      | dataSet(5).name = 'Roll 0.2 Hz IA'
      | dataSet(6).timeRange = [0 60]
      | dataSet(6).name = 'Roll 0.1 Hz IA'
      | dataSet(7).timeRange = [0 60]
      | dataSet(7).name = 'Roll 0.05 Hz IA'
      | dataSet(8).timeRange = [0 60]
      | dataSet(8).name = 'Roll 0.2 Hz RC'
      | dataSet(9).timeRange = [0 60]
      | dataSet(9).name = 'Roll 0.1 Hz RC'
      | dataSet(10).timeRange = [0 60]
      | dataSet(10).name = 'Roll 0.05 Hz RC'
      | dataSet(11).timeRange = [0 60]
      | dataSet(11).name = 'SimpleSims'
      | dataSet(12).timeRange = [0 60]
      | dataSet(12).name = 'YawOKN30degs'
      | sbobj.Groups(1).Name = 'Zeros'
      | sbobj.Groups(1).Signals(1).Name = 'N-O (roll)'
      | sbobj.Groups(1).Signals(1).XData = [0 60]
      | sbobj.Groups(1).Signals(1).YData = [0 0]
      | sbobj.Groups(1).Signals(2).Name = 'I-A (pitch)'
      | sbobj.Groups(1).Signals(2).XData = [0 60]
      | sbobj.Groups(1).Signals(2).YData = [0 0]
      | sbobj.Groups(1).Signals(3).Name = 'R-C (yaw)'
      | sbobj.Groups(1).Signals(3).XData = [0 60]
      | sbobj.Groups(1).Signals(3).YData = [0 0]
      | sbobj.Groups(1).TimeRange = [0 60]
      | sbobj.Groups(2).Name = 'Roll 0.2 Hz'
      | sbobj.Groups(2).Signals(1).Name = 'N-O (roll)'
      | sbobj.Groups(2).Signals(1).XData = [0 0.00500500500501 0.01001001001 0.015015015015 0.02002002002 0.025025025025 0.03003003003 0.035035035035 0.04004004004 0.045045045045 0.0500500500501 0.0550550550551 ... (11989 elements, 1x11989)]
      | sbobj.Groups(2).Signals(1).YData = [0 0.125788666321 0.251572356775 0.377346095689 0.503104907788 0.628843818382 0.754557853574 0.880242040448 1.00589140727 1.13150098368 1.25706580089 1.3825808919 ... (11989 elements, 1x11989)]
      | sbobj.Groups(2).Signals(2).Name = 'I-A (pitch)'
      | sbobj.Groups(2).Signals(2).XData = [0 60]
      | sbobj.Groups(2).Signals(2).YData = [0 0]
      | sbobj.Groups(2).Signals(3).Name = 'R-C (yaw)'
      | sbobj.Groups(2).Signals(3).XData = [0 60]
      | sbobj.Groups(2).Signals(3).YData = [0 0]
      | sbobj.Groups(2).TimeRange = [0 60]
      | sbobj.Groups(3).Name = 'Roll 0.1 Hz'
      | sbobj.Groups(3).Signals(1).Name = 'N-O (roll)'
      | sbobj.Groups(3).Signals(1).XData = [0 0.01001001001 0.02002002002 0.03003003003 0.04004004004 0.0500500500501 0.0600600600601 0.0700700700701 0.0800800800801 0.0900900900901 0.1001001001 0.11011011011 ... (5995 elements, 1x5995)]
      | sbobj.Groups(3).Signals(1).YData = [0 0.125788666321 0.251572356775 0.377346095689 0.503104907788 0.628843818382 0.754557853574 0.880242040448 1.00589140727 1.13150098368 1.25706580089 1.3825808919 ... (5995 elements, 1x5995)]
      | sbobj.Groups(3).Signals(2).Name = 'I-A (pitch)'
      | sbobj.Groups(3).Signals(2).XData = [0 60]
      | sbobj.Groups(3).Signals(2).YData = [0 0]
      | sbobj.Groups(3).Signals(3).Name = 'R-C (yaw)'
      | sbobj.Groups(3).Signals(3).XData = [0 60]
      | sbobj.Groups(3).Signals(3).YData = [0 0]
      | sbobj.Groups(3).TimeRange = [0 60]
      | sbobj.Groups(4).Name = 'Roll 0.05 Hz'
      | sbobj.Groups(4).Signals(1).Name = 'N-O (roll)'
      | sbobj.Groups(4).Signals(1).XData = [0 0.02002002002 0.04004004004 0.0600600600601 0.0800800800801 0.1001001001 0.12012012012 0.14014014014 0.16016016016 0.18018018018 0.2002002002 0.22022022022 ... (2998 elements, 1x2998)]
      | sbobj.Groups(4).Signals(1).YData = [0 0.125788666321 0.251572356775 0.377346095689 0.503104907788 0.628843818382 0.754557853574 0.880242040448 1.00589140727 1.13150098368 1.25706580089 1.3825808919 ... (2998 elements, 1x2998)]
      | sbobj.Groups(4).Signals(2).Name = 'I-A (pitch)'
      | sbobj.Groups(4).Signals(2).XData = [0 60]
      | sbobj.Groups(4).Signals(2).YData = [0 0]
      | sbobj.Groups(4).Signals(3).Name = 'R-C (yaw)'
      | sbobj.Groups(4).Signals(3).XData = [0 60]
      | sbobj.Groups(4).Signals(3).YData = [0 0]
      | sbobj.Groups(4).TimeRange = [0 60]
      | sbobj.Groups(5).Name = 'Roll 0.2 Hz IA'
      | sbobj.Groups(5).Signals(1).Name = 'N-O (roll)'
      | sbobj.Groups(5).Signals(1).XData = [0 60]
      | sbobj.Groups(5).Signals(1).YData = [0 0]
      | sbobj.Groups(5).Signals(2).Name = 'I-A (pitch)'
      | sbobj.Groups(5).Signals(2).XData = [0 0.00500500500501 0.01001001001 0.015015015015 0.02002002002 0.025025025025 0.03003003003 0.035035035035 0.04004004004 0.045045045045 0.0500500500501 0.0550550550551 ... (11989 elements, 1x11989)]
      | sbobj.Groups(5).Signals(2).YData = [0 0.125788666321 0.251572356775 0.377346095689 0.503104907788 0.628843818382 0.754557853574 0.880242040448 1.00589140727 1.13150098368 1.25706580089 1.3825808919 ... (11989 elements, 1x11989)]
      | sbobj.Groups(5).Signals(3).Name = 'R-C (yaw)'
      | sbobj.Groups(5).Signals(3).XData = [0 60]
      | sbobj.Groups(5).Signals(3).YData = [0 0]
      | sbobj.Groups(5).TimeRange = [0 60]
      | sbobj.Groups(6).Name = 'Roll 0.1 Hz IA'
      | sbobj.Groups(6).Signals(1).Name = 'N-O (roll)'
      | sbobj.Groups(6).Signals(1).XData = [0 60]
      | sbobj.Groups(6).Signals(1).YData = [0 0]
      | sbobj.Groups(6).Signals(2).Name = 'I-A (pitch)'
      | sbobj.Groups(6).Signals(2).XData = [0 0.01001001001 0.02002002002 0.03003003003 0.04004004004 0.0500500500501 0.0600600600601 0.0700700700701 0.0800800800801 0.0900900900901 0.1001001001 0.11011011011 ... (5995 elements, 1x5995)]
      | sbobj.Groups(6).Signals(2).YData = [0 0.125788666321 0.251572356775 0.377346095689 0.503104907788 0.628843818382 0.754557853574 0.880242040448 1.00589140727 1.13150098368 1.25706580089 1.3825808919 ... (5995 elements, 1x5995)]
      | sbobj.Groups(6).Signals(3).Name = 'R-C (yaw)'
      | sbobj.Groups(6).Signals(3).XData = [0 60]
      | sbobj.Groups(6).Signals(3).YData = [0 0]
      | sbobj.Groups(6).TimeRange = [0 60]
      | sbobj.Groups(7).Name = 'Roll 0.05 Hz IA'
      | sbobj.Groups(7).Signals(1).Name = 'N-O (roll)'
      | sbobj.Groups(7).Signals(1).XData = [0 60]
      | sbobj.Groups(7).Signals(1).YData = [0 0]
      | sbobj.Groups(7).Signals(2).Name = 'I-A (pitch)'
      | sbobj.Groups(7).Signals(2).XData = [0 0.02002002002 0.04004004004 0.0600600600601 0.0800800800801 0.1001001001 0.12012012012 0.14014014014 0.16016016016 0.18018018018 0.2002002002 0.22022022022 ... (2998 elements, 1x2998)]
      | sbobj.Groups(7).Signals(2).YData = [0 0.125788666321 0.251572356775 0.377346095689 0.503104907788 0.628843818382 0.754557853574 0.880242040448 1.00589140727 1.13150098368 1.25706580089 1.3825808919 ... (2998 elements, 1x2998)]
      | sbobj.Groups(7).Signals(3).Name = 'R-C (yaw)'
      | sbobj.Groups(7).Signals(3).XData = [0 60]
      | sbobj.Groups(7).Signals(3).YData = [0 0]
      | sbobj.Groups(7).TimeRange = [0 60]
      | sbobj.Groups(8).Name = 'Roll 0.2 Hz RC'
      | sbobj.Groups(8).Signals(1).Name = 'N-O (roll)'
      | sbobj.Groups(8).Signals(1).XData = [0 60]
      | sbobj.Groups(8).Signals(1).YData = [0 0]
      | sbobj.Groups(8).Signals(2).Name = 'I-A (pitch)'
      | sbobj.Groups(8).Signals(2).XData = [0 60]
      | sbobj.Groups(8).Signals(2).YData = [0 0]
      | sbobj.Groups(8).Signals(3).Name = 'R-C (yaw)'
      | sbobj.Groups(8).Signals(3).XData = [0 0.00500500500501 0.01001001001 0.015015015015 0.02002002002 0.025025025025 0.03003003003 0.035035035035 0.04004004004 0.045045045045 0.0500500500501 0.0550550550551 ... (11989 elements, 1x11989)]
      | sbobj.Groups(8).Signals(3).YData = [0 0.125788666321 0.251572356775 0.377346095689 0.503104907788 0.628843818382 0.754557853574 0.880242040448 1.00589140727 1.13150098368 1.25706580089 1.3825808919 ... (11989 elements, 1x11989)]
      | sbobj.Groups(8).TimeRange = [0 60]
      | sbobj.Groups(9).Name = 'Roll 0.1 Hz RC'
      | sbobj.Groups(9).Signals(1).Name = 'N-O (roll)'
      | sbobj.Groups(9).Signals(1).XData = [0 60]
      | sbobj.Groups(9).Signals(1).YData = [0 0]
      | sbobj.Groups(9).Signals(2).Name = 'I-A (pitch)'
      | sbobj.Groups(9).Signals(2).XData = [0 60]
      | sbobj.Groups(9).Signals(2).YData = [0 0]
      | sbobj.Groups(9).Signals(3).Name = 'R-C (yaw)'
      | sbobj.Groups(9).Signals(3).XData = [0 0.01001001001 0.02002002002 0.03003003003 0.04004004004 0.0500500500501 0.0600600600601 0.0700700700701 0.0800800800801 0.0900900900901 0.1001001001 0.11011011011 ... (5995 elements, 1x5995)]
      | sbobj.Groups(9).Signals(3).YData = [0 0.125788666321 0.251572356775 0.377346095689 0.503104907788 0.628843818382 0.754557853574 0.880242040448 1.00589140727 1.13150098368 1.25706580089 1.3825808919 ... (5995 elements, 1x5995)]
      | sbobj.Groups(9).TimeRange = [0 60]
      | sbobj.Groups(10).Name = 'Roll 0.05 Hz RC'
      | sbobj.Groups(10).Signals(1).Name = 'N-O (roll)'
      | sbobj.Groups(10).Signals(1).XData = [0 60]
      | sbobj.Groups(10).Signals(1).YData = [0 0]
      | sbobj.Groups(10).Signals(2).Name = 'I-A (pitch)'
      | sbobj.Groups(10).Signals(2).XData = [0 60]
      | sbobj.Groups(10).Signals(2).YData = [0 0]
      | sbobj.Groups(10).Signals(3).Name = 'R-C (yaw)'
      | sbobj.Groups(10).Signals(3).XData = [0 0.02002002002 0.04004004004 0.0600600600601 0.0800800800801 0.1001001001 0.12012012012 0.14014014014 0.16016016016 0.18018018018 0.2002002002 0.22022022022 ... (2998 elements, 1x2998)]
      | sbobj.Groups(10).Signals(3).YData = [0 0.125788666321 0.251572356775 0.377346095689 0.503104907788 0.628843818382 0.754557853574 0.880242040448 1.00589140727 1.13150098368 1.25706580089 1.3825808919 ... (2998 elements, 1x2998)]
      | sbobj.Groups(10).TimeRange = [0 60]
      | sbobj.Groups(11).Name = 'SimpleSims'
      | sbobj.Groups(11).Signals(1).Name = 'N-O (roll)'
      | sbobj.Groups(11).Signals(1).XData = [0 0.01 0.02 0.03 0.04 0.05 0.06 0.07 0.08 0.09 0.1 0.11 ... (6001 elements, 1x6001)]
      | sbobj.Groups(11).Signals(1).YData = [0 0.0628317497176 0.125662879311 0.188492768663 0.251320797667 0.314146346236 0.376968794308 0.43978752185 0.502601908867 0.565411335405 0.628215181563 0.691012827489 ... (6001 elements, 1x6001)]
      | sbobj.Groups(11).Signals(2).Name = 'I-A (pitch)'
      | sbobj.Groups(11).Signals(2).XData = [0 5 35 60]
      | sbobj.Groups(11).Signals(2).YData = [0 0 0 0]
      | sbobj.Groups(11).Signals(3).Name = 'R-C (yaw)'
      | sbobj.Groups(11).Signals(3).XData = [0 5 35 60]
      | sbobj.Groups(11).Signals(3).YData = [0 0 0 0]
      | sbobj.Groups(11).TimeRange = [0 60]
      | sbobj.Groups(12).Name = 'YawOKN30degs'
      | sbobj.Groups(12).Signals(1).Name = 'N-O (roll)'
      | sbobj.Groups(12).Signals(1).XData = [0 60]
      | sbobj.Groups(12).Signals(1).YData = [0 0]
      | sbobj.Groups(12).Signals(2).Name = 'I-A (pitch)'
      | sbobj.Groups(12).Signals(2).XData = [0 60]
      | sbobj.Groups(12).Signals(2).YData = [0 0]
      | sbobj.Groups(12).Signals(3).Name = 'R-C (yaw)'
      | sbobj.Groups(12).Signals(3).XData = [0 10 10 40.05 40.05 60]
      | sbobj.Groups(12).Signals(3).YData = [0 0 30 30 0 0]
      | sbobj.Groups(12).TimeRange = [0 60]
  Subsystem : Subsystem
  Bus : Outport
  wires:
  FromWs/1 -> Subsystem/1(In1)
  Subsystem/1(N-O (roll)) -> Bus Creator/1  "N-O (roll)"
  Subsystem/2(I-A (pitch)) -> Bus Creator/2  "I-A (pitch)"
  Subsystem/3(R-C (yaw)) -> Bus Creator/3  "R-C (yaw)"
  Bus Creator/1 -> Bus/1

== system OcularMotorLabModel_2024_01_02_M21b/Visual World Intrinsic velocity ==
  Bus Creator : BusCreator  Tag=Bus Creator  Inputs=3
  FromWs : FromWorkspace  Tag=STV FromWs  VariableName=tuvar
      SigBuilderData=|
      | common.afterFinalStr = 'Extrapolate'
      | common.sampleTime = 0
      | dataSet(1).timeRange = [0 60]
      | dataSet(1).name = 'Zeros'
      | dataSet(2).timeRange = [0 60]
      | dataSet(2).name = 'Roll 0.2 Hz'
      | dataSet(3).timeRange = [0 60]
      | dataSet(3).name = 'Roll 0.1 Hz'
      | dataSet(4).timeRange = [0 60]
      | dataSet(4).name = 'Roll 0.05 Hz'
      | dataSet(5).timeRange = [0 60]
      | dataSet(5).name = 'Roll 0.2 Hz IA'
      | dataSet(6).timeRange = [0 60]
      | dataSet(6).name = 'Roll 0.1 Hz IA'
      | dataSet(7).timeRange = [0 60]
      | dataSet(7).name = 'Roll 0.05 Hz IA'
      | dataSet(8).timeRange = [0 60]
      | dataSet(8).name = 'Roll 0.2 Hz RC'
      | dataSet(9).timeRange = [0 60]
      | dataSet(9).name = 'Roll 0.1 Hz RC'
      | dataSet(10).timeRange = [0 60]
      | dataSet(10).name = 'Roll 0.05 Hz RC'
      | dataSet(11).timeRange = [0 60]
      | dataSet(11).name = 'SimpleSims'
      | dataSet(12).timeRange = [0 60]
      | dataSet(12).name = 'YawOKN30degs'
      | sbobj.Groups(1).Name = 'Zeros'
      | sbobj.Groups(1).Signals(1).Name = 'N-O (roll)'
      | sbobj.Groups(1).Signals(1).XData = [0 60]
      | sbobj.Groups(1).Signals(1).YData = [0 0]
      | sbobj.Groups(1).Signals(2).Name = 'I-A (pitch)'
      | sbobj.Groups(1).Signals(2).XData = [0 60]
      | sbobj.Groups(1).Signals(2).YData = [0 0]
      | sbobj.Groups(1).Signals(3).Name = 'R-C (yaw)'
      | sbobj.Groups(1).Signals(3).XData = [0 60]
      | sbobj.Groups(1).Signals(3).YData = [0 0]
      | sbobj.Groups(1).TimeRange = [0 60]
      | sbobj.Groups(2).Name = 'Roll 0.2 Hz'
      | sbobj.Groups(2).Signals(1).Name = 'N-O (roll)'
      | sbobj.Groups(2).Signals(1).XData = [0 0.00500500500501 0.01001001001 0.015015015015 0.02002002002 0.025025025025 0.03003003003 0.035035035035 0.04004004004 0.045045045045 0.0500500500501 0.0550550550551 ... (11989 elements, 1x11989)]
      | sbobj.Groups(2).Signals(1).YData = [0 0.125788666321 0.251572356775 0.377346095689 0.503104907788 0.628843818382 0.754557853574 0.880242040448 1.00589140727 1.13150098368 1.25706580089 1.3825808919 ... (11989 elements, 1x11989)]
      | sbobj.Groups(2).Signals(2).Name = 'I-A (pitch)'
      | sbobj.Groups(2).Signals(2).XData = [0 60]
      | sbobj.Groups(2).Signals(2).YData = [0 0]
      | sbobj.Groups(2).Signals(3).Name = 'R-C (yaw)'
      | sbobj.Groups(2).Signals(3).XData = [0 60]
      | sbobj.Groups(2).Signals(3).YData = [0 0]
      | sbobj.Groups(2).TimeRange = [0 60]
      | sbobj.Groups(3).Name = 'Roll 0.1 Hz'
      | sbobj.Groups(3).Signals(1).Name = 'N-O (roll)'
      | sbobj.Groups(3).Signals(1).XData = [0 0.01001001001 0.02002002002 0.03003003003 0.04004004004 0.0500500500501 0.0600600600601 0.0700700700701 0.0800800800801 0.0900900900901 0.1001001001 0.11011011011 ... (5995 elements, 1x5995)]
      | sbobj.Groups(3).Signals(1).YData = [0 0.125788666321 0.251572356775 0.377346095689 0.503104907788 0.628843818382 0.754557853574 0.880242040448 1.00589140727 1.13150098368 1.25706580089 1.3825808919 ... (5995 elements, 1x5995)]
      | sbobj.Groups(3).Signals(2).Name = 'I-A (pitch)'
      | sbobj.Groups(3).Signals(2).XData = [0 60]
      | sbobj.Groups(3).Signals(2).YData = [0 0]
      | sbobj.Groups(3).Signals(3).Name = 'R-C (yaw)'
      | sbobj.Groups(3).Signals(3).XData = [0 60]
      | sbobj.Groups(3).Signals(3).YData = [0 0]
      | sbobj.Groups(3).TimeRange = [0 60]
      | sbobj.Groups(4).Name = 'Roll 0.05 Hz'
      | sbobj.Groups(4).Signals(1).Name = 'N-O (roll)'
      | sbobj.Groups(4).Signals(1).XData = [0 0.02002002002 0.04004004004 0.0600600600601 0.0800800800801 0.1001001001 0.12012012012 0.14014014014 0.16016016016 0.18018018018 0.2002002002 0.22022022022 ... (2998 elements, 1x2998)]
      | sbobj.Groups(4).Signals(1).YData = [0 0.125788666321 0.251572356775 0.377346095689 0.503104907788 0.628843818382 0.754557853574 0.880242040448 1.00589140727 1.13150098368 1.25706580089 1.3825808919 ... (2998 elements, 1x2998)]
      | sbobj.Groups(4).Signals(2).Name = 'I-A (pitch)'
      | sbobj.Groups(4).Signals(2).XData = [0 60]
      | sbobj.Groups(4).Signals(2).YData = [0 0]
      | sbobj.Groups(4).Signals(3).Name = 'R-C (yaw)'
      | sbobj.Groups(4).Signals(3).XData = [0 60]
      | sbobj.Groups(4).Signals(3).YData = [0 0]
      | sbobj.Groups(4).TimeRange = [0 60]
      | sbobj.Groups(5).Name = 'Roll 0.2 Hz IA'
      | sbobj.Groups(5).Signals(1).Name = 'N-O (roll)'
      | sbobj.Groups(5).Signals(1).XData = [0 60]
      | sbobj.Groups(5).Signals(1).YData = [0 0]
      | sbobj.Groups(5).Signals(2).Name = 'I-A (pitch)'
      | sbobj.Groups(5).Signals(2).XData = [0 0.00500500500501 0.01001001001 0.015015015015 0.02002002002 0.025025025025 0.03003003003 0.035035035035 0.04004004004 0.045045045045 0.0500500500501 0.0550550550551 ... (11989 elements, 1x11989)]
      | sbobj.Groups(5).Signals(2).YData = [0 0.125788666321 0.251572356775 0.377346095689 0.503104907788 0.628843818382 0.754557853574 0.880242040448 1.00589140727 1.13150098368 1.25706580089 1.3825808919 ... (11989 elements, 1x11989)]
      | sbobj.Groups(5).Signals(3).Name = 'R-C (yaw)'
      | sbobj.Groups(5).Signals(3).XData = [0 60]
      | sbobj.Groups(5).Signals(3).YData = [0 0]
      | sbobj.Groups(5).TimeRange = [0 60]
      | sbobj.Groups(6).Name = 'Roll 0.1 Hz IA'
      | sbobj.Groups(6).Signals(1).Name = 'N-O (roll)'
      | sbobj.Groups(6).Signals(1).XData = [0 60]
      | sbobj.Groups(6).Signals(1).YData = [0 0]
      | sbobj.Groups(6).Signals(2).Name = 'I-A (pitch)'
      | sbobj.Groups(6).Signals(2).XData = [0 0.01001001001 0.02002002002 0.03003003003 0.04004004004 0.0500500500501 0.0600600600601 0.0700700700701 0.0800800800801 0.0900900900901 0.1001001001 0.11011011011 ... (5995 elements, 1x5995)]
      | sbobj.Groups(6).Signals(2).YData = [0 0.125788666321 0.251572356775 0.377346095689 0.503104907788 0.628843818382 0.754557853574 0.880242040448 1.00589140727 1.13150098368 1.25706580089 1.3825808919 ... (5995 elements, 1x5995)]
      | sbobj.Groups(6).Signals(3).Name = 'R-C (yaw)'
      | sbobj.Groups(6).Signals(3).XData = [0 60]
      | sbobj.Groups(6).Signals(3).YData = [0 0]
      | sbobj.Groups(6).TimeRange = [0 60]
      | sbobj.Groups(7).Name = 'Roll 0.05 Hz IA'
      | sbobj.Groups(7).Signals(1).Name = 'N-O (roll)'
      | sbobj.Groups(7).Signals(1).XData = [0 60]
      | sbobj.Groups(7).Signals(1).YData = [0 0]
      | sbobj.Groups(7).Signals(2).Name = 'I-A (pitch)'
      | sbobj.Groups(7).Signals(2).XData = [0 0.02002002002 0.04004004004 0.0600600600601 0.0800800800801 0.1001001001 0.12012012012 0.14014014014 0.16016016016 0.18018018018 0.2002002002 0.22022022022 ... (2998 elements, 1x2998)]
      | sbobj.Groups(7).Signals(2).YData = [0 0.125788666321 0.251572356775 0.377346095689 0.503104907788 0.628843818382 0.754557853574 0.880242040448 1.00589140727 1.13150098368 1.25706580089 1.3825808919 ... (2998 elements, 1x2998)]
      | sbobj.Groups(7).Signals(3).Name = 'R-C (yaw)'
      | sbobj.Groups(7).Signals(3).XData = [0 60]
      | sbobj.Groups(7).Signals(3).YData = [0 0]
      | sbobj.Groups(7).TimeRange = [0 60]
      | sbobj.Groups(8).Name = 'Roll 0.2 Hz RC'
      | sbobj.Groups(8).Signals(1).Name = 'N-O (roll)'
      | sbobj.Groups(8).Signals(1).XData = [0 60]
      | sbobj.Groups(8).Signals(1).YData = [0 0]
      | sbobj.Groups(8).Signals(2).Name = 'I-A (pitch)'
      | sbobj.Groups(8).Signals(2).XData = [0 60]
      | sbobj.Groups(8).Signals(2).YData = [0 0]
      | sbobj.Groups(8).Signals(3).Name = 'R-C (yaw)'
      | sbobj.Groups(8).Signals(3).XData = [0 0.00500500500501 0.01001001001 0.015015015015 0.02002002002 0.025025025025 0.03003003003 0.035035035035 0.04004004004 0.045045045045 0.0500500500501 0.0550550550551 ... (11989 elements, 1x11989)]
      | sbobj.Groups(8).Signals(3).YData = [0 0.125788666321 0.251572356775 0.377346095689 0.503104907788 0.628843818382 0.754557853574 0.880242040448 1.00589140727 1.13150098368 1.25706580089 1.3825808919 ... (11989 elements, 1x11989)]
      | sbobj.Groups(8).TimeRange = [0 60]
      | sbobj.Groups(9).Name = 'Roll 0.1 Hz RC'
      | sbobj.Groups(9).Signals(1).Name = 'N-O (roll)'
      | sbobj.Groups(9).Signals(1).XData = [0 60]
      | sbobj.Groups(9).Signals(1).YData = [0 0]
      | sbobj.Groups(9).Signals(2).Name = 'I-A (pitch)'
      | sbobj.Groups(9).Signals(2).XData = [0 60]
      | sbobj.Groups(9).Signals(2).YData = [0 0]
      | sbobj.Groups(9).Signals(3).Name = 'R-C (yaw)'
      | sbobj.Groups(9).Signals(3).XData = [0 0.01001001001 0.02002002002 0.03003003003 0.04004004004 0.0500500500501 0.0600600600601 0.0700700700701 0.0800800800801 0.0900900900901 0.1001001001 0.11011011011 ... (5995 elements, 1x5995)]
      | sbobj.Groups(9).Signals(3).YData = [0 0.125788666321 0.251572356775 0.377346095689 0.503104907788 0.628843818382 0.754557853574 0.880242040448 1.00589140727 1.13150098368 1.25706580089 1.3825808919 ... (5995 elements, 1x5995)]
      | sbobj.Groups(9).TimeRange = [0 60]
      | sbobj.Groups(10).Name = 'Roll 0.05 Hz RC'
      | sbobj.Groups(10).Signals(1).Name = 'N-O (roll)'
      | sbobj.Groups(10).Signals(1).XData = [0 60]
      | sbobj.Groups(10).Signals(1).YData = [0 0]
      | sbobj.Groups(10).Signals(2).Name = 'I-A (pitch)'
      | sbobj.Groups(10).Signals(2).XData = [0 60]
      | sbobj.Groups(10).Signals(2).YData = [0 0]
      | sbobj.Groups(10).Signals(3).Name = 'R-C (yaw)'
      | sbobj.Groups(10).Signals(3).XData = [0 0.02002002002 0.04004004004 0.0600600600601 0.0800800800801 0.1001001001 0.12012012012 0.14014014014 0.16016016016 0.18018018018 0.2002002002 0.22022022022 ... (2998 elements, 1x2998)]
      | sbobj.Groups(10).Signals(3).YData = [0 0.125788666321 0.251572356775 0.377346095689 0.503104907788 0.628843818382 0.754557853574 0.880242040448 1.00589140727 1.13150098368 1.25706580089 1.3825808919 ... (2998 elements, 1x2998)]
      | sbobj.Groups(10).TimeRange = [0 60]
      | sbobj.Groups(11).Name = 'SimpleSims'
      | sbobj.Groups(11).Signals(1).Name = 'N-O (roll)'
      | sbobj.Groups(11).Signals(1).XData = [0 0.01 0.02 0.03 0.04 0.05 0.06 0.07 0.08 0.09 0.1 0.11 ... (6001 elements, 1x6001)]
      | sbobj.Groups(11).Signals(1).YData = [0 0.0628317497176 0.125662879311 0.188492768663 0.251320797667 0.314146346236 0.376968794308 0.43978752185 0.502601908867 0.565411335405 0.628215181563 0.691012827489 ... (6001 elements, 1x6001)]
      | sbobj.Groups(11).Signals(2).Name = 'I-A (pitch)'
      | sbobj.Groups(11).Signals(2).XData = [0 5 35 60]
      | sbobj.Groups(11).Signals(2).YData = [0 0 0 0]
      | sbobj.Groups(11).Signals(3).Name = 'R-C (yaw)'
      | sbobj.Groups(11).Signals(3).XData = [0 5 35 60]
      | sbobj.Groups(11).Signals(3).YData = [0 0 0 0]
      | sbobj.Groups(11).TimeRange = [0 60]
      | sbobj.Groups(12).Name = 'YawOKN30degs'
      | sbobj.Groups(12).Signals(1).Name = 'N-O (roll)'
      | sbobj.Groups(12).Signals(1).XData = [0 60]
      | sbobj.Groups(12).Signals(1).YData = [0 0]
      | sbobj.Groups(12).Signals(2).Name = 'I-A (pitch)'
      | sbobj.Groups(12).Signals(2).XData = [0 60]
      | sbobj.Groups(12).Signals(2).YData = [0 0]
      | sbobj.Groups(12).Signals(3).Name = 'R-C (yaw)'
      | sbobj.Groups(12).Signals(3).XData = [0 10 10 40.05 40.05 60]
      | sbobj.Groups(12).Signals(3).YData = [0 0 30 30 0 0]
      | sbobj.Groups(12).TimeRange = [0 60]
  Subsystem : Subsystem
  Bus : Outport
  wires:
  FromWs/1 -> Subsystem/1(In1)
  Subsystem/1(N-O (roll)) -> Bus Creator/1  "N-O (roll)"
  Subsystem/2(I-A (pitch)) -> Bus Creator/2  "I-A (pitch)"
  Subsystem/3(R-C (yaw)) -> Bus Creator/3  "R-C (yaw)"
  Bus Creator/1 -> Bus/1

== system OcularMotorLabModel_2024_01_02_M21b/Visual linear world extrinsic velocity ==
  Bus Creator : BusCreator  Tag=Bus Creator  Inputs=3
  FromWs : FromWorkspace  Tag=STV FromWs  VariableName=tuvar
      SigBuilderData=|
      | common.afterFinalStr = 'Extrapolate'
      | common.sampleTime = 0
      | dataSet(1).timeRange = [0 40]
      | dataSet(1).name = 'Zeros'
      | dataSet(2).timeRange = [0 60]
      | dataSet(2).name = 'Sample Sims'
      | dataSet(3).timeRange = [0 40]
      | dataSet(3).name = 'Translate forward'
      | sbobj.Groups(1).Name = 'Zeros'
      | sbobj.Groups(1).Signals(1).Name = 'vx'
      | sbobj.Groups(1).Signals(1).XData = [0 5 6 15 40]
      | sbobj.Groups(1).Signals(1).YData = [0 0 0 0 0]
      | sbobj.Groups(1).Signals(2).Name = 'vy'
      | sbobj.Groups(1).Signals(2).XData = [0 5 6 40]
      | sbobj.Groups(1).Signals(2).YData = [0 0 0 0]
      | sbobj.Groups(1).Signals(3).Name = 'vz'
      | sbobj.Groups(1).Signals(3).XData = [0 5 15 40]
      | sbobj.Groups(1).Signals(3).YData = [0 0 0 0]
      | sbobj.Groups(1).TimeRange = [0 40]
      | sbobj.Groups(2).Name = 'Sample Sims'
      | sbobj.Groups(2).Signals(1).Name = 'vx'
      | sbobj.Groups(2).Signals(1).XData = [0 5 60]
      | sbobj.Groups(2).Signals(1).YData = [0 0 0]
      | sbobj.Groups(2).Signals(2).Name = 'vy'
      | sbobj.Groups(2).Signals(2).XData = [0 5 35 60]
      | sbobj.Groups(2).Signals(2).YData = [0 0 0 0]
      | sbobj.Groups(2).Signals(3).Name = 'vz'
      | sbobj.Groups(2).Signals(3).XData = [0 20.05 20.05 50.05 50.05 60]
      | sbobj.Groups(2).Signals(3).YData = [0 0 -30 -30 0 0]
      | sbobj.Groups(2).TimeRange = [0 60]
      | sbobj.Groups(3).Name = 'Translate forward'
      | sbobj.Groups(3).Signals(1).Name = 'vx'
      | sbobj.Groups(3).Signals(1).XData = [0 5 5 6 6 40]
      | sbobj.Groups(3).Signals(1).YData = [0 0 0.81 0.81 0 0]
      | sbobj.Groups(3).Signals(2).Name = 'vy'
      | sbobj.Groups(3).Signals(2).XData = [0 5 6 40]
      | sbobj.Groups(3).Signals(2).YData = [0 0 0 0]
      | sbobj.Groups(3).Signals(3).Name = 'vz'
      | sbobj.Groups(3).Signals(3).XData = [0 5 15 40]
      | sbobj.Groups(3).Signals(3).YData = [0 0 0 0]
      | sbobj.Groups(3).TimeRange = [0 40]
  Subsystem : Subsystem
  Bus : Outport
  wires:
  FromWs/1 -> Subsystem/1(In1)
  Subsystem/1(vx) -> Bus Creator/1  "vx"
  Subsystem/2(vy) -> Bus Creator/2  "vy"
  Subsystem/3(vz) -> Bus Creator/3  "vz"
  Bus Creator/1 -> Bus/1

== system OcularMotorLabModel_2024_01_02_M21b/Visual linear world intrinsic velocity ==
  Bus Creator : BusCreator  Tag=Bus Creator  Inputs=3
  FromWs : FromWorkspace  Tag=STV FromWs  VariableName=tuvar
      SigBuilderData=|
      | common.afterFinalStr = 'Extrapolate'
      | common.sampleTime = 0
      | dataSet(1).timeRange = [0 40]
      | dataSet(1).name = 'Zeros'
      | dataSet(2).timeRange = [0 60]
      | dataSet(2).name = 'Sample Sims'
      | dataSet(3).timeRange = [0 40]
      | dataSet(3).name = 'Translate forward'
      | sbobj.Groups(1).Name = 'Zeros'
      | sbobj.Groups(1).Signals(1).Name = 'vX'
      | sbobj.Groups(1).Signals(1).XData = [0 5 6 15 40]
      | sbobj.Groups(1).Signals(1).YData = [0 0 0 0 0]
      | sbobj.Groups(1).Signals(2).Name = 'vY'
      | sbobj.Groups(1).Signals(2).XData = [0 5 6 40]
      | sbobj.Groups(1).Signals(2).YData = [0 0 0 0]
      | sbobj.Groups(1).Signals(3).Name = 'vZ'
      | sbobj.Groups(1).Signals(3).XData = [0 5 15 40]
      | sbobj.Groups(1).Signals(3).YData = [0 0 0 0]
      | sbobj.Groups(1).TimeRange = [0 40]
      | sbobj.Groups(2).Name = 'Sample Sims'
      | sbobj.Groups(2).Signals(1).Name = 'vX'
      | sbobj.Groups(2).Signals(1).XData = [0 5 60]
      | sbobj.Groups(2).Signals(1).YData = [0 0 0]
      | sbobj.Groups(2).Signals(2).Name = 'vY'
      | sbobj.Groups(2).Signals(2).XData = [0 5 35 60]
      | sbobj.Groups(2).Signals(2).YData = [0 0 0 0]
      | sbobj.Groups(2).Signals(3).Name = 'vZ'
      | sbobj.Groups(2).Signals(3).XData = [0 20.05 20.05 50.05 50.05 60]
      | sbobj.Groups(2).Signals(3).YData = [0 0 -30 -30 0 0]
      | sbobj.Groups(2).TimeRange = [0 60]
      | sbobj.Groups(3).Name = 'Translate forward'
      | sbobj.Groups(3).Signals(1).Name = 'vX'
      | sbobj.Groups(3).Signals(1).XData = [0 5 5 6 6 40]
      | sbobj.Groups(3).Signals(1).YData = [0 0 0.81 0.81 0 0]
      | sbobj.Groups(3).Signals(2).Name = 'vY'
      | sbobj.Groups(3).Signals(2).XData = [0 5 6 40]
      | sbobj.Groups(3).Signals(2).YData = [0 0 0 0]
      | sbobj.Groups(3).Signals(3).Name = 'vZ'
      | sbobj.Groups(3).Signals(3).XData = [0 5 15 40]
      | sbobj.Groups(3).Signals(3).YData = [0 0 0 0]
      | sbobj.Groups(3).TimeRange = [0 40]
  Subsystem : Subsystem
  Bus : Outport
  wires:
  FromWs/1 -> Subsystem/1(In1)
  Subsystem/1(vX) -> Bus Creator/1  "vX"
  Subsystem/2(vY) -> Bus Creator/2  "vY"
  Subsystem/3(vZ) -> Bus Creator/3  "vZ"
  Bus Creator/1 -> Bus/1

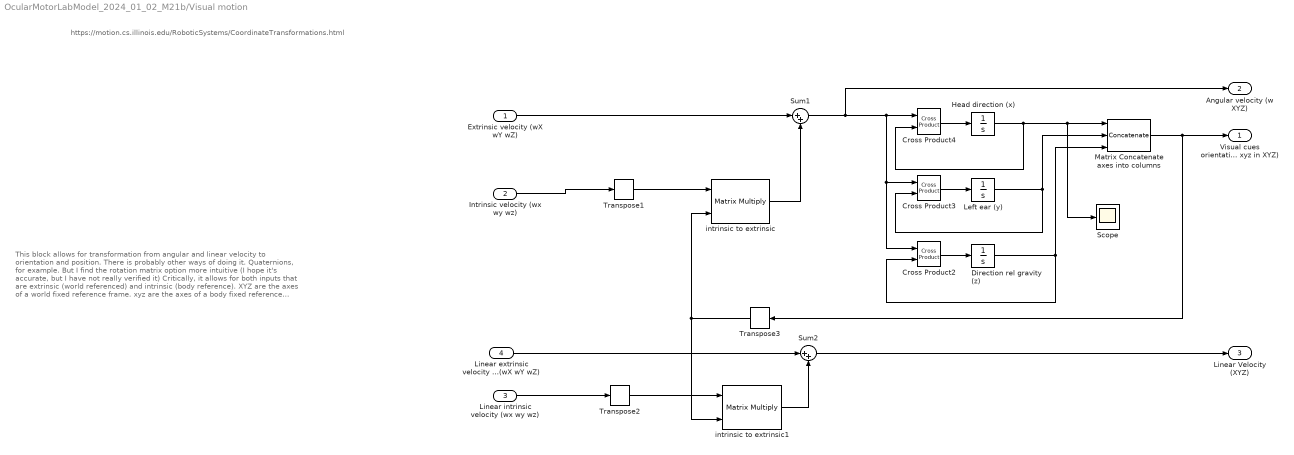
== system OcularMotorLabModel_2024_01_02_M21b/Visual motion ==
  note: https://motion.cs.illinois.edu/RoboticSystems/CoordinateTransformations.html
  note: This block allows for transformation from angular and linear velocity to orientation and position. There is probably other ways of doing it. Quaternions, for example. But I find the rotation matrix option more intuitive (I hope it's accurate, but I have not really verified it)
      |
      | Critically, it allows for both inputs that are extrinsic (world referenced) and intrinsic (body reference).
      |
      | XYZ are the axes of a world fixed reference frame.
      | xyz are the axes of a body fixed reference frame
      |
      | For the extrinsic angular velocities, they need to be integrated after a cross product with each of the xyz axis, that way they provide the rotation of such axis within the XYZ world fixed reference frame.
      |
      | For the intrinsic angular velocities, they simply multiply each of the intrisic axis and get added to the extrinsic velocities.
      |
      | A similar approach is followed for the linear velocities but without the cross products are linear velocities can be simply integrated by components.
  Extrinsic velocity (wX wY wZ) : Inport
  Intrinsic velocity (wx wy wz) : Inport  Port=2
  Linear intrinsic velocity (wx wy wz) : Inport  Port=3
  Linear extrinsic velocity (wX wY wZ) : Inport  Port=4
  Cross Product2 : vrlib/Utilities/Cross Product
  Cross Product3 : vrlib/Utilities/Cross Product
  Cross Product4 : vrlib/Utilities/Cross Product
  Direction rel gravity (z) : Integrator  InitialCondition=[0 0 1]
  Head direction (x) : Integrator  InitialCondition=[1 0 0]
  Left ear (y) : Integrator  InitialCondition=[0 1 0]
  Matrix Concatenate axes into columns : Concatenate  NumInputs=3  Mode=Multidimensional array  ConcatenateDimension=2
  Scope : Scope
  Sum1 : Sum  Inputs=|++
  Sum2 : Sum  Inputs=|++
  Transpose1 : matrix_library/Transpose
  Transpose2 : matrix_library/Transpose
  Transpose3 : matrix_library/Transpose
  intrinsic to extrinsic : Product  Multiplication=Matrix(*)
  intrinsic to extrinsic1 : Product  Multiplication=Matrix(*)
  Visual cues orientation in world (R xyz in XYZ) : Outport
  Angular velocity (w XYZ) : Outport  Port=2
  Linear Velocity (XYZ) : Outport  Port=3
  wires:
  Matrix Concatenate axes into columns/1 -> Visual cues orientation in world (R xyz in XYZ)/1, Transpose3/1
  Linear intrinsic velocity (wx wy wz)/1 -> Transpose2/1
  Transpose2/1 -> intrinsic to extrinsic1/1
  Transpose1/1 -> intrinsic to extrinsic/1
  Intrinsic velocity (wx wy wz)/1 -> Transpose1/1
  Transpose3/1 -> intrinsic to extrinsic1/2, intrinsic to extrinsic/2
  Cross Product2/1 -> Direction rel gravity (z)/1
  Linear extrinsic velocity (wX wY wZ)/1 -> Sum2/1
  intrinsic to extrinsic1/1 -> Sum2/2
  Sum2/1 -> Linear Velocity (XYZ)/1
  Cross Product3/1 -> Left ear (y)/1
  Extrinsic velocity (wX wY wZ)/1 -> Sum1/1
  Sum1/1 -> Angular velocity (w XYZ)/1, Cross Product2/1, Cross Product3/1, Cross Product4/1
  intrinsic to extrinsic/1 -> Sum1/2
  Left ear (y)/1 -> Matrix Concatenate axes into columns/2, Cross Product3/2
  Direction rel gravity (z)/1 -> Matrix Concatenate axes into columns/3, Cross Product2/2
  Head direction (x)/1 -> Scope/1, Matrix Concatenate axes into columns/1, Cross Product4/2
  Cross Product4/1 -> Head direction (x)/1

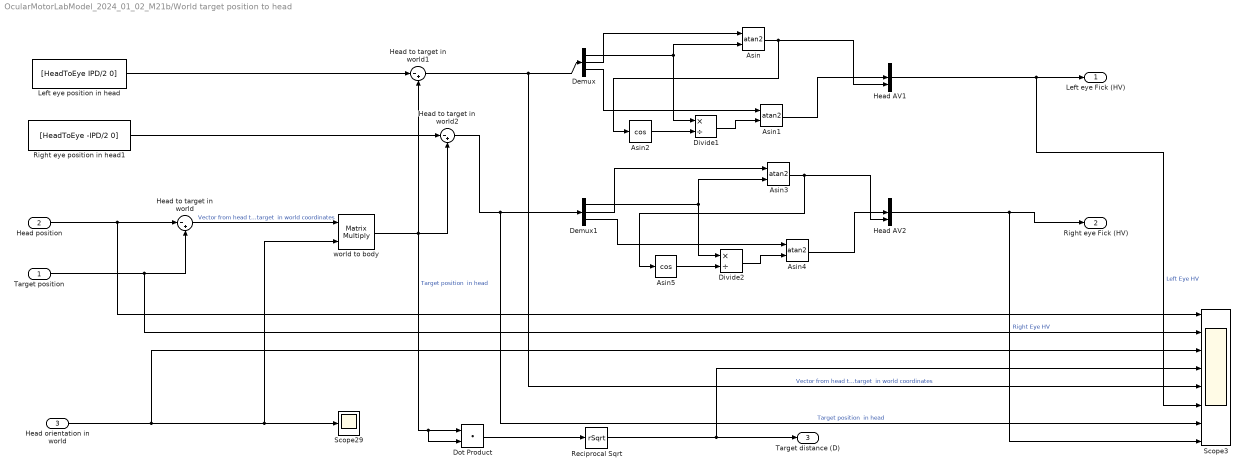
== system OcularMotorLabModel_2024_01_02_M21b/World target position to head ==
  Target position : Inport
  Head position : Inport  Port=2
  Head orientation in world : Inport  Port=3
  Asin{,1,3..4} (4 alike) : Trigonometry  Operator=atan2
  Asin2 : Trigonometry  Operator=cos
  Asin5 : Trigonometry  Operator=cos
  Demux : Demux  Outputs=3
  Demux1 : Demux  Outputs=3
  Divide1 : Product  Inputs=*/
  Divide2 : Product  Inputs=*/
  Dot Product : DotProduct  InputSameDT=on  OutDataTypeStr=Inherit: Inherit via internal rule
  Head AV1 : Mux  Inputs=3
  Head AV2 : Mux  Inputs=3
  Head to target in world : Sum  Inputs=|-+
  Head to target in world1 : Sum  Inputs=|-+
  Head to target in world2 : Sum  Inputs=|-+
  Left eye position in head : Constant  Value=[HeadToEye IPD/2 0]
  Reciprocal Sqrt : Sqrt  Operator=rSqrt  SaturateOnIntegerOverflow=on
  Right eye position in head1 : Constant  Value=[HeadToEye -IPD/2 0]
  Scope29 : Scope
  Scope3 : Scope  NumInputPorts=8
  world to body : Product  Multiplication=Matrix(*)
  Left eye Fick (HV) : Outport
  Right eye Fick (HV) : Outport  Port=2
  Target distance (D) : Outport  Port=3
  wires:
  world to body/1 -> Head to target in world1/2, Head to target in world2/2, Dot Product/2, Dot Product/1  "Target position  in head"
  Target position/1 -> Scope3/2, Head to target in world/2
  Head position/1 -> Scope3/1, Head to target in world/1
  Head to target in world/1 -> world to body/1  "Vector from head to target  in world coordinates"
  Head orientation in world/1 -> Scope3/3, world to body/2, Scope29/1
  Dot Product/1 -> Reciprocal Sqrt/1
  Reciprocal Sqrt/1 -> Scope3/4, Target distance (D)/1
  Head AV1/1 -> Scope3/6, Left eye Fick (HV)/1  "Left Eye HV"
  Head to target in world1/1 -> Scope3/5, Demux/1  "Vector from head to target  in world coordinates"
  Head AV2/1 -> Scope3/8, Right eye Fick (HV)/1  "Right Eye HV"
  Right eye position in head1/1 -> Head to target in world2/1
  Demux/1 -> Asin/2, Divide1/1
  Demux/2 -> Asin/1
  Asin/1 -> Head AV1/3, Asin2/1
  Asin1/1 -> Head AV1/2
  Demux/3 -> Asin1/1
  Divide1/1 -> Asin1/2
  Asin2/1 -> Divide1/2
  Divide2/1 -> Asin4/2
  Demux1/2 -> Asin3/1
  Demux1/1 -> Asin3/2, Divide2/1
  Asin4/1 -> Head AV2/2
  Asin3/1 -> Head AV2/3, Asin5/1
  Asin5/1 -> Divide2/2
  Demux1/3 -> Asin4/1
  Head to target in world2/1 -> Scope3/7, Demux1/1  "Target position  in head"
  Left eye position in head/1 -> Head to target in world1/1

== system OcularMotorLabModel_2024_01_02_M21b/World to head ==
  note: GIa is calculated as the vector sum of G and linear acceleration in body reference
  Orientation : Inport
  Linear acceleration : Inport  Port=2
  1/G : Gain  Gain=1/9.8
  G (XYZ) : Constant  Value=[0 0 -1]  VectorParams1D=off
  Rotate gravity to body coordinates : Product  Multiplication=Matrix(*)
  Rotate gravity to body coordinates1 : Product  Multiplication=Matrix(*)
  Sum : Sum  Inputs=++|
  Transpose1 : matrix_library/Transpose
  Transpose2 : matrix_library/Transpose
  GIA (in Gs) : Outport
  wires:
  Orientation/1 -> Rotate gravity to body coordinates/2, Rotate gravity to body coordinates1/2
  Rotate gravity to body coordinates/1 -> Transpose1/1
  G (XYZ)/1 -> Rotate gravity to body coordinates/1
  Sum/1 -> GIA (in Gs)/1  "GIA"
  1/G/1 -> Rotate gravity to body coordinates1/1
  Rotate gravity to body coordinates1/1 -> Transpose2/1
  Linear acceleration/1 -> 1/G/1
  Transpose1/1 -> Sum/1
  Transpose2/1 -> Sum/2

== system OcularMotorLabModel_2024_01_02_M21b/World to head  ==
  Head orientation : Inport
  Head velocity : Inport  Port=2
  world to body : Product  Multiplication=Matrix(*)
  Head velocity1 : Outport
  wires:
  Head orientation/1 -> world to body/2
  Head velocity/1 -> world to body/1
  world to body/1 -> Head velocity1/1

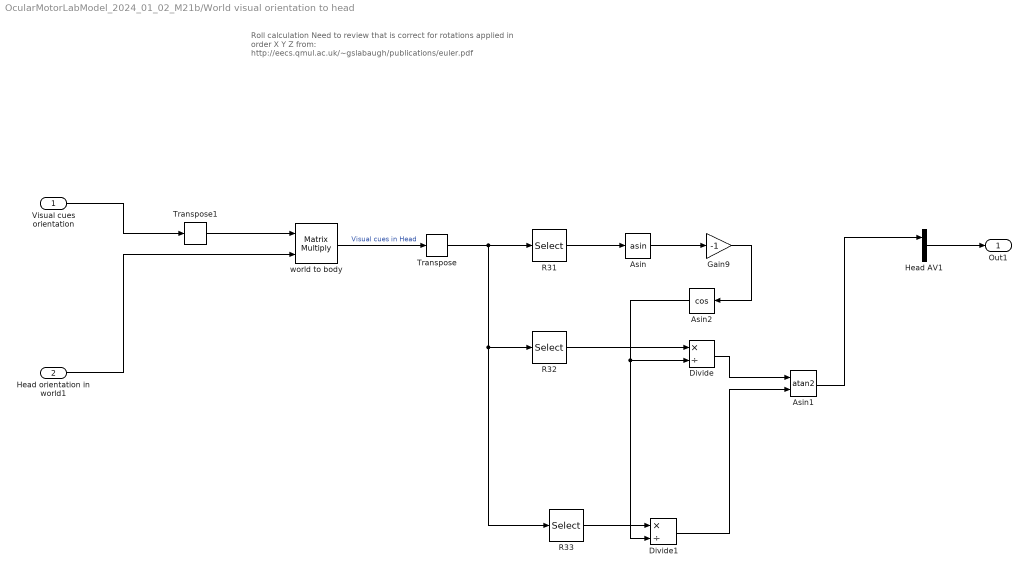
== system OcularMotorLabModel_2024_01_02_M21b/World visual orientation to head ==
  note: Roll calculation
      |
      | Need to review that is correct for rotations applied in order X Y Z
      |
      | from: http://eecs.qmul.ac.uk/~gslabaugh/publications/euler.pdf
  Visual cues orientation : Inport
  Head orientation in world1 : Inport  Port=2
  Asin : Trigonometry  Operator=asin
  Asin1 : Trigonometry  Operator=atan2
  Asin2 : Trigonometry  Operator=cos
  Divide : Product  Inputs=*/
  Divide1 : Product  Inputs=*/
  Gain9 : Gain  Gain=-1
  Head AV1 : Mux  Inputs=3
  R31 : Selector  NumberOfDimensions=2  InputPortWidth=3  IndexOptions=Index vector (dialog),Index vector (dialog)  Indices=3,1  OutputSizes=1,1
  R32 : Selector  NumberOfDimensions=2  InputPortWidth=3  IndexOptions=Index vector (dialog),Index vector (dialog)  Indices=3,2  OutputSizes=1,1
  R33 : Selector  NumberOfDimensions=2  InputPortWidth=3  IndexOptions=Index vector (dialog),Index vector (dialog)  Indices=3,3  OutputSizes=1,1
  Transpose : matrix_library/Transpose
  Transpose1 : matrix_library/Transpose
  world to body : Product  Multiplication=Matrix(*)
  Out1 : Outport
  wires:
  Transpose/1 -> R31/1, R32/1, R33/1
  world to body/1 -> Transpose/1  "Visual cues in Head"
  Visual cues orientation/1 -> Transpose1/1
  Head orientation in world1/1 -> world to body/2
  Gain9/1 -> Asin2/1
  Asin1/1 -> Head AV1/1
  Head AV1/1 -> Out1/1
  R31/1 -> Asin/1
  R32/1 -> Divide/1
  Asin/1 -> Gain9/1
  R33/1 -> Divide1/1
  Divide1/1 -> Asin1/2
  Divide/1 -> Asin1/1
  Transpose1/1 -> world to body/1
  Asin2/1 -> Divide1/2, Divide/2

== system OcularMotorLabModel_2024_01_02_M21b/World visual velocity  to head ==
  Visual velocity in world : Inport
  Head velocity in world : Inport  Port=2
  Head orientation in world : Inport  Port=3
  Transpose : matrix_library/Transpose
  visual velocity : Sum  Inputs=|+-
  world to body : Product  Multiplication=Matrix(*)
  Visual velocity in Head : Outport
  wires:
  Head orientation in world/1 -> world to body/2
  Visual velocity in world/1 -> visual velocity/1
  world to body/1 -> Transpose/1
  visual velocity/1 -> world to body/1
  Transpose/1 -> Visual velocity in Head/1  "Visual velocity in Head"
  Head velocity in world/1 -> visual velocity/2

== system OcularMotorLabModel_2024_01_02_M21b/Head velocity (body)/Subsystem ==
  In1 : Inport
  Demux : Demux  Tag=STV Demux  Outputs=3
      settings: DisplayOption=none
  nasooccipital : Outport  Tag=STV Outport
  interaural : Outport  Tag=STV Outport  Port=2
  rostrocaudal : Outport  Tag=STV Outport  Port=3
  wires:
  Demux/1 -> nasooccipital/1
  Demux/2 -> interaural/1
  Demux/3 -> rostrocaudal/1
  In1/1 -> Demux/1

== system OcularMotorLabModel_2024_01_02_M21b/Head velocity (world)/Subsystem ==
  In1 : Inport
  Demux : Demux  Tag=STV Demux  Outputs=3
      settings: DisplayOption=none
  x : Outport  Tag=STV Outport
  y : Outport  Tag=STV Outport  Port=2
  z : Outport  Tag=STV Outport  Port=3
  wires:
  Demux/1 -> x/1
  Demux/2 -> y/1
  Demux/3 -> z/1
  In1/1 -> Demux/1

== system OcularMotorLabModel_2024_01_02_M21b/Linear body velocity/Subsystem ==
  In1 : Inport
  Demux : Demux  Tag=STV Demux  Outputs=3
      settings: DisplayOption=none
  vx : Outport  Tag=STV Outport
  vy : Outport  Tag=STV Outport  Port=2
  vz : Outport  Tag=STV Outport  Port=3
  wires:
  Demux/1 -> vx/1
  Demux/2 -> vy/1
  Demux/3 -> vz/1
  In1/1 -> Demux/1

== system OcularMotorLabModel_2024_01_02_M21b/Linear world velocity/Subsystem ==
  In1 : Inport
  Demux : Demux  Tag=STV Demux  Outputs=3
      settings: DisplayOption=none
  vX : Outport  Tag=STV Outport
  vY : Outport  Tag=STV Outport  Port=2
  vZ : Outport  Tag=STV Outport  Port=3
  wires:
  Demux/1 -> vX/1
  Demux/2 -> vY/1
  Demux/3 -> vZ/1
  In1/1 -> Demux/1

== system OcularMotorLabModel_2024_01_02_M21b/Only for simulations of spv/Left eye plant1 ==
  In1 : Inport
  Demux : Demux  Outputs=3
  Mux : Mux  Inputs=3
  Plant1 : TransferFcn  Numerator=[Tz 1]  Denominator=[T1*T2 (T1+T2) 1]
  Plant2 : TransferFcn  Numerator=[w^2]  Denominator=[1 + 2*psi*w w^2]
  Plant3 : TransferFcn  Numerator=[Tz 1]  Denominator=[T1*T2 (T1+T2) 1]
  Plant4 : TransferFcn  Numerator=[w^2]  Denominator=[1 + 2*psi*w w^2]
  Plant5 : TransferFcn  Numerator=[Tz 1]  Denominator=[T1*T2 (T1+T2) 1]
  Plant6 : TransferFcn  Numerator=[w^2]  Denominator=[1 + 2*psi*w w^2]
  Saturation : Saturate  UpperLimit=50*pi/180  LowerLimit=-50*pi/180
  Eye position : Outport
  wires:
  In1/1 -> Demux/1
  Mux/1 -> Saturation/1  "Eye position"
  Plant4/1 -> Mux/1
  Plant2/1 -> Mux/2
  Plant6/1 -> Mux/3
  Demux/1 -> Plant3/1
  Demux/2 -> Plant1/1
  Demux/3 -> Plant5/1
  Saturation/1 -> Eye position/1
  Plant3/1 -> Plant4/1
  Plant1/1 -> Plant2/1
  Plant5/1 -> Plant6/1

== system OcularMotorLabModel_2024_01_02_M21b/Pursuit velocity corollary/Eye plant ==
  In1 : Inport
  Demux : Demux  Outputs=3
  Mux : Mux  Inputs=3
  Plant1 : TransferFcn  Numerator=[Tz 1]  Denominator=[T1*T2 (T1+T2) 1]
  Plant2 : TransferFcn  Numerator=[w^2]  Denominator=[1 + 2*psi*w w^2]
  Plant3 : TransferFcn  Numerator=[Tz 1]  Denominator=[T1*T2 (T1+T2) 1]
  Plant4 : TransferFcn  Numerator=[w^2]  Denominator=[1 + 2*psi*w w^2]
  Plant5 : TransferFcn  Numerator=[Tz 1]  Denominator=[T1*T2 (T1+T2) 1]
  Plant6 : TransferFcn  Numerator=[w^2]  Denominator=[1 + 2*psi*w w^2]
  Eye position : Outport
  wires:
  In1/1 -> Demux/1
  Mux/1 -> Eye position/1  "Eye position"
  Plant4/1 -> Mux/1
  Plant2/1 -> Mux/2
  Plant6/1 -> Mux/3
  Demux/1 -> Plant3/1
  Demux/2 -> Plant1/1
  Demux/3 -> Plant5/1
  Plant3/1 -> Plant4/1
  Plant1/1 -> Plant2/1
  Plant5/1 -> Plant6/1

== system OcularMotorLabModel_2024_01_02_M21b/Saccade velocity corollary/Eye plant ==
  In1 : Inport
  Demux : Demux  Outputs=3
  Mux : Mux  Inputs=3
  Plant1 : TransferFcn  Numerator=[Tz 1]  Denominator=[T1*T2 (T1+T2) 1]
  Plant2 : TransferFcn  Numerator=[w^2]  Denominator=[1 + 2*psi*w w^2]
  Plant3 : TransferFcn  Numerator=[Tz 1]  Denominator=[T1*T2 (T1+T2) 1]
  Plant4 : TransferFcn  Numerator=[w^2]  Denominator=[1 + 2*psi*w w^2]
  Plant5 : TransferFcn  Numerator=[Tz 1]  Denominator=[T1*T2 (T1+T2) 1]
  Plant6 : TransferFcn  Numerator=[w^2]  Denominator=[1 + 2*psi*w w^2]
  Eye position : Outport
  wires:
  In1/1 -> Demux/1
  Mux/1 -> Eye position/1  "Eye position"
  Plant4/1 -> Mux/1
  Plant2/1 -> Mux/2
  Plant6/1 -> Mux/3
  Demux/1 -> Plant3/1
  Demux/2 -> Plant1/1
  Demux/3 -> Plant5/1
  Plant3/1 -> Plant4/1
  Plant1/1 -> Plant2/1
  Plant5/1 -> Plant6/1

== system OcularMotorLabModel_2024_01_02_M21b/Smooth pursuit/Acceleration saturation ==
  In1 : Inport
  Gain2 : Gain  Gain=Asp1
  Gain3 : Gain  Gain=Asp2
  Saturation1 : Saturate  UpperLimit=deg2rad(e0sp)  LowerLimit=-deg2rad(e0sp)
  Sum2 : Sum  Inputs=++|
  Out1 : Outport
  wires:
  In1/1 -> Saturation1/1, Gain3/1
  Saturation1/1 -> Gain2/1
  Sum2/1 -> Out1/1
  Gain3/1 -> Sum2/2
  Gain2/1 -> Sum2/1

== system OcularMotorLabModel_2024_01_02_M21b/Smooth pursuit/Internal model ==
  note: It's important for this internal model to not have a leaky integrator. Otherwise a positive feedback loop is created with retinal motion that it is not discounted but amplified post saccades.
      |
      | Haven't fully grasped it and there are still questions about the plant and the slide. But for now this seems to work ok.
  note: Gaze holding integrator
  Corollary input : Inport
  Demux2 : Demux  Outputs=3
  Direct : Gain  Gain=Gpc
  Eye plant : Subsystem
  Integrator1 : Integrator
  "MN " : Sum  Inputs=+++  InputSameDT=on  SaturateOnIntegerOverflow=on  OutDataTypeStr=Inherit: Same as first input
  Mux2 : Mux  Inputs=3
  Position bias6 : TransferFcn  Numerator=[Gsl]  Denominator=[Tsl 1]
  Position bias7 : TransferFcn  Numerator=[Gsl]  Denominator=[Tsl 1]
  Position bias8 : TransferFcn  Numerator=[Gsl]  Denominator=[Tsl 1]
  Eye position : Outport
  wires:
  Demux2/2 -> Position bias7/1
  Mux2/1 -> "MN "/3
  Position bias8/1 -> Mux2/3
  Demux2/3 -> Position bias8/1
  Direct/1 -> "MN "/2
  Demux2/1 -> Position bias6/1
  Position bias6/1 -> Mux2/1
  Integrator1/1 -> "MN "/1
  Corollary input/1 -> Demux2/1, Direct/1, Integrator1/1
  "MN "/1 -> Eye plant/1(In1)  "Corollary integrator"
  Position bias7/1 -> Mux2/2
  Eye plant/1(Eye position) -> Eye position/1  "Eye position"

== system OcularMotorLabModel_2024_01_02_M21b/Target position/Subsystem ==
  In1 : Inport
  Demux : Demux  Tag=STV Demux  Outputs=3
      settings: DisplayOption=none
  tX (m - postiive forward) : Outport  Tag=STV Outport  VectorParamsAs1DForOutWhenUnconnected=off
  tY (m - postive to left) : Outport  Tag=STV Outport  Port=2  VectorParamsAs1DForOutWhenUnconnected=off
  tZ (m - positive up) : Outport  Tag=STV Outport  Port=3  VectorParamsAs1DForOutWhenUnconnected=off
  wires:
  Demux/1 -> tX (m - postiive forward)/1
  Demux/2 -> tY (m - postive to left)/1
  Demux/3 -> tZ (m - positive up)/1
  In1/1 -> Demux/1

== system OcularMotorLabModel_2024_01_02_M21b/Vergence (distance) corollary/Eye plant ==
  Motor output : Inport
  Plant5 : TransferFcn  Numerator=[Tz 1]  Denominator=[T1*T2 (T1+T2) 1]
  Plant6 : TransferFcn  Numerator=[w^2]  Denominator=[1 + 2*psi*w w^2]
  Eye position : Outport
  wires:
  Plant5/1 -> Plant6/1
  Motor output/1 -> Plant5/1
  Plant6/1 -> Eye position/1

== system OcularMotorLabModel_2024_01_02_M21b/Version Position corollary/Eye plant ==
  Motor output : Inport
  Demux : Demux  Outputs=3
  Mux : Mux  Inputs=3
  Plant1 : TransferFcn  Numerator=[Tz 1]  Denominator=[T1*T2 (T1+T2) 1]
  Plant2 : TransferFcn  Numerator=[w^2]  Denominator=[1 + 2*psi*w w^2]
  Plant3 : TransferFcn  Numerator=[Tz 1]  Denominator=[T1*T2 (T1+T2) 1]
  Plant4 : TransferFcn  Numerator=[w^2]  Denominator=[1 + 2*psi*w w^2]
  Plant5 : TransferFcn  Numerator=[Tz 1]  Denominator=[T1*T2 (T1+T2) 1]
  Plant6 : TransferFcn  Numerator=[w^2]  Denominator=[1 + 2*psi*w w^2]
  Eye position : Outport
  wires:
  Motor output/1 -> Demux/1
  Mux/1 -> Eye position/1  "Eye position"
  Plant4/1 -> Mux/1
  Plant2/1 -> Mux/2
  Plant6/1 -> Mux/3
  Demux/1 -> Plant3/1
  Demux/2 -> Plant1/1
  Demux/3 -> Plant5/1
  Plant3/1 -> Plant4/1
  Plant1/1 -> Plant2/1
  Plant5/1 -> Plant6/1

== system OcularMotorLabModel_2024_01_02_M21b/Visual World Extrinsic Orientation/Subsystem ==
  In1 : Inport
  Demux : Demux  Tag=STV Demux  Outputs=3
      settings: DisplayOption=none
  N-O (roll) : Outport  Tag=STV Outport
  I-A (pitch) : Outport  Tag=STV Outport  Port=2
  R-C (yaw) : Outport  Tag=STV Outport  Port=3
  wires:
  Demux/1 -> N-O (roll)/1
  Demux/2 -> I-A (pitch)/1
  Demux/3 -> R-C (yaw)/1
  In1/1 -> Demux/1

== system OcularMotorLabModel_2024_01_02_M21b/Visual World Extrinsic velocity/Subsystem ==
  In1 : Inport
  Demux : Demux  Tag=STV Demux  Outputs=3
      settings: DisplayOption=none
  N-O (roll) : Outport  Tag=STV Outport
  I-A (pitch) : Outport  Tag=STV Outport  Port=2
  R-C (yaw) : Outport  Tag=STV Outport  Port=3
  wires:
  Demux/1 -> N-O (roll)/1
  Demux/2 -> I-A (pitch)/1
  Demux/3 -> R-C (yaw)/1
  In1/1 -> Demux/1

== system OcularMotorLabModel_2024_01_02_M21b/Visual World Intrinsic velocity/Subsystem ==
  In1 : Inport
  Demux : Demux  Tag=STV Demux  Outputs=3
      settings: DisplayOption=none
  N-O (roll) : Outport  Tag=STV Outport
  I-A (pitch) : Outport  Tag=STV Outport  Port=2
  R-C (yaw) : Outport  Tag=STV Outport  Port=3
  wires:
  Demux/1 -> N-O (roll)/1
  Demux/2 -> I-A (pitch)/1
  Demux/3 -> R-C (yaw)/1
  In1/1 -> Demux/1

== system OcularMotorLabModel_2024_01_02_M21b/Visual linear world extrinsic velocity/Subsystem ==
  In1 : Inport
  Demux : Demux  Tag=STV Demux  Outputs=3
      settings: DisplayOption=none
  vx : Outport  Tag=STV Outport
  vy : Outport  Tag=STV Outport  Port=2
  vz : Outport  Tag=STV Outport  Port=3
  wires:
  Demux/1 -> vx/1
  Demux/2 -> vy/1
  Demux/3 -> vz/1
  In1/1 -> Demux/1

== system OcularMotorLabModel_2024_01_02_M21b/Visual linear world intrinsic velocity/Subsystem ==
  In1 : Inport
  Demux : Demux  Tag=STV Demux  Outputs=3
      settings: DisplayOption=none
  vX : Outport  Tag=STV Outport
  vY : Outport  Tag=STV Outport  Port=2
  vZ : Outport  Tag=STV Outport  Port=3
  wires:
  Demux/1 -> vX/1
  Demux/2 -> vY/1
  Demux/3 -> vZ/1
  In1/1 -> Demux/1

== system OcularMotorLabModel_2024_01_02_M21b/Smooth pursuit/Internal model/Eye plant ==
  In1 : Inport
  Demux : Demux  Outputs=3
  Mux : Mux  Inputs=3
  Plant1 : TransferFcn  Numerator=[Tz 1]  Denominator=[T1*T2 (T1+T2) 1]
  Plant2 : TransferFcn  Numerator=[w^2]  Denominator=[1 + 2*psi*w w^2]
  Plant3 : TransferFcn  Numerator=[Tz 1]  Denominator=[T1*T2 (T1+T2) 1]
  Plant4 : TransferFcn  Numerator=[w^2]  Denominator=[1 + 2*psi*w w^2]
  Plant5 : TransferFcn  Numerator=[Tz 1]  Denominator=[T1*T2 (T1+T2) 1]
  Plant6 : TransferFcn  Numerator=[w^2]  Denominator=[1 + 2*psi*w w^2]
  Eye position : Outport
  wires:
  In1/1 -> Demux/1
  Mux/1 -> Eye position/1  "Eye position"
  Plant4/1 -> Mux/1
  Plant2/1 -> Mux/2
  Plant6/1 -> Mux/3
  Demux/1 -> Plant3/1
  Demux/2 -> Plant1/1
  Demux/3 -> Plant5/1
  Plant3/1 -> Plant4/1
  Plant1/1 -> Plant2/1
  Plant5/1 -> Plant6/1
